simulink model "ForwardKinematic_YuMi"  (R2024a)
(part 11 of 23)

(7514214926474921*cos(q2L)*((6384186990310915*cos(q1L))/9007199254740992 + (5557241208790345*sin(q1L))/9007199254740992))/36893488147419103232 - sin(q2L)*((5557241208790345*cos(q1L))/9007199254740992 - (6384186990310915*sin(q1L))/9007199254740992)))/9007199254740992 - (1764482024691522628700660907665*sin(q3L)*((55491554575214198102159220722265*sin(q2L))/162259276829213363391578010288128 + cos(q2L)*((5557241208790345*cos(q1L))/9007199254740992 - (6384186990310915*sin(q1L))/9007199254740992) + (7514214926474921*sin(q2L)*((6384186990310915*cos(q1L))/9007199254740992 + (5557241208790345*sin(q1L))/9007199254740992))/36893488147419103232))/42535295865117307932921825928971026432))/9007199254740992))/36893488147419103232000 - (33294932745128518861295532433359*cos(q2L))/3245185536584267267831560205762560 - (81*((9007199067919185*cos(q4L))/9007199254740992 - (234819211581865*sin(q4L))/1152921504606846976)*((499823478647255911063139966257565597426350154025*sin(q2L))/1461501637330902918203684832716283019655932542976 + (9007199067919185*cos(q2L)*((5557241208790345*cos(q1L))/9007199254740992 - (6384186990310915*sin(q1L))/9007199254740992))/9007199254740992 + (67682029681889335677290557259385*sin(q2L)*((6384186990310915*cos(q1L))/9007199254740992 + (5557241208790345*sin(q1L))/9007199254740992))/332306998946228968225951765070086144))/2000 + (81222263116692158804177042061221826384594597321566869716687*((234819211581865*cos(q4L))/1152921504606846976 + (9007199067919185*sin(q4L))/9007199254740992)*((499823478647255911063139966257565597426350154025*sin(q2L))/1461501637330902918203684832716283019655932542976 + (9007199067919185*cos(q2L)*((5557241208790345*cos(q1L))/9007199254740992 - (6384186990310915*sin(q1L))/9007199254740992))/9007199254740992 + (67682029681889335677290557259385*sin(q2L)*((6384186990310915*cos(q1L))/9007199254740992 + (5557241208790345*sin(q1L))/9007199254740992))/332306998946228968225951765070086144))/306499108173177771671669405430061836723747824436720435200000 - (324259171862923063*sin(q6L)*((9007199067919185*sin(q5L)*((783310804561232573774573497517025067305577458842146606386579375*sin(q2L))/55213970774324510299478046898216203619608871777363092441300193790394368 + (14115856197532180673579726082375*cos(q2L)*((5557241208790345*cos(q1L))/9007199254740992 - (6384186990310915*sin(q1L))/9007199254740992))/340282366920938463463374607431768211456 + (106069577339469832923929692356850887620017617375*sin(q2L)*((6384186990310915*cos(q1L))/9007199254740992 + (5557241208790345*sin(q1L))/9007199254740992))/12554203470773361527671578846415332832204710888928069025792 - (234819211581865*cos(q3L)*((55491554575214198102159220722265*cos(q2L))/162259276829213363391578010288128 + (7514214926474921*cos(q2L)*((6384186990310915*cos(q1L))/9007199254740992 + (5557241208790345*sin(q1L))/9007199254740992))/36893488147419103232 - sin(q2L)*((5557241208790345*cos(q1L))/9007199254740992 - (6384186990310915*sin(q1L))/9007199254740992)))/1152921504606846976 + (67682029681889335677290557259385*cos(q3L)*((55491554575214198102159220722265*sin(q2L))/162259276829213363391578010288128 + cos(q2L)*((5557241208790345*cos(q1L))/9007199254740992 - (6384186990310915*sin(q1L))/9007199254740992) + (7514214926474921*sin(q2L)*((6384186990310915*cos(q1L))/9007199254740992 + (5557241208790345*sin(q1L))/9007199254740992))/36893488147419103232))/332306998946228968225951765070086144 - (9007199067919185*sin(q3L)*((55491554575214198102159220722265*cos(q2L))/162259276829213363391578010288128 + (7514214926474921*cos(q2L)*((6384186990310915*cos(q1L))/9007199254740992 + (5557241208790345*sin(q1L))/9007199254740992))/36893488147419103232 - sin(q2L)*((5557241208790345*cos(q1L))/9007199254740992 - (6384186990310915*sin(q1L))/9007199254740992)))/9007199254740992 - (1764482024691522628700660907665*sin(q3L)*((55491554575214198102159220722265*sin(q2L))/162259276829213363391578010288128 + cos(q2L)*((5557241208790345*cos(q1L))/9007199254740992 - (6384186990310915*sin(q1L))/9007199254740992) + (7514214926474921*sin(q2L)*((6384186990310915*cos(q1L))/9007199254740992 + (5557241208790345*sin(q1L))/9007199254740992))/36893488147419103232))/42535295865117307932921825928971026432))/9007199254740992 - cos(q5L)*(((9007199067919185*cos(q4L))/9007199254740992 - (234819211581865*sin(q4L))/1152921504606846976)*((499823478647255911063139966257565597426350154025*sin(q2L))/1461501637330902918203684832716283019655932542976 + (9007199067919185*cos(q2L)*((5557241208790345*cos(q1L))/9007199254740992 - (6384186990310915*sin(q1L))/9007199254740992))/9007199254740992 + (67682029681889335677290557259385*sin(q2L)*((6384186990310915*cos(q1L))/9007199254740992 + (5557241208790345*sin(q1L))/9007199254740992))/332306998946228968225951765070086144) + (7514214926474921*sin(q4L)*((7514214926474921*cos(q3L)*((55491554575214198102159220722265*sin(q2L))/162259276829213363391578010288128 + cos(q2L)*((5557241208790345*cos(q1L))/9007199254740992 - (6384186990310915*sin(q1L))/9007199254740992) + (7514214926474921*sin(q2L)*((6384186990310915*cos(q1L))/9007199254740992 + (5557241208790345*sin(q1L))/9007199254740992))/36893488147419103232))/36893488147419103232 - sin(q3L)*((55491554575214198102159220722265*cos(q2L))/162259276829213363391578010288128 + (7514214926474921*cos(q2L)*((6384186990310915*cos(q1L))/9007199254740992 + (5557241208790345*sin(q1L))/9007199254740992))/36893488147419103232 - sin(q2L)*((5557241208790345*cos(q1L))/9007199254740992 - (6384186990310915*sin(q1L))/9007199254740992))))/36893488147419103232 + (cos(q3L)*((55491554575214198102159220722265*cos(q2L))/162259276829213363391578010288128 + (7514214926474921*cos(q2L)*((6384186990310915*cos(q1L))/9007199254740992 + (5557241208790345*sin(q1L))/9007199254740992))/36893488147419103232 - sin(q2L)*((5557241208790345*cos(q1L))/9007199254740992 - (6384186990310915*sin(q1L))/9007199254740992)) + (7514214926474921*sin(q3L)*((55491554575214198102159220722265*sin(q2L))/162259276829213363391578010288128 + cos(q2L)*((5557241208790345*cos(q1L))/9007199254740992 - (6384186990310915*sin(q1L))/9007199254740992) + (7514214926474921*sin(q2L)*((6384186990310915*cos(q1L))/9007199254740992 + (5557241208790345*sin(q1L))/9007199254740992))/36893488147419103232))/36893488147419103232)*((7514214926474921*cos(q4L))/36893488147419103232 + (4503599440548691*sin(q4L))/4503599627370496)) + (7514214926474921*sin(q5L)*((7514214926474921*cos(q4L)*((7514214926474921*cos(q3L)*((55491554575214198102159220722265*sin(q2L))/162259276829213363391578010288128 + cos(q2L)*((5557241208790345*cos(q1L))/9007199254740992 - (6384186990310915*sin(q1L))/9007199254740992) + (7514214926474921*sin(q2L)*((6384186990310915*cos(q1L))/9007199254740992 + (5557241208790345*sin(q1L))/9007199254740992))/36893488147419103232))/36893488147419103232 - sin(q3L)*((55491554575214198102159220722265*cos(q2L))/162259276829213363391578010288128 + (7514214926474921*cos(q2L)*((6384186990310915*cos(q1L))/9007199254740992 + (5557241208790345*sin(q1L))/9007199254740992))/36893488147419103232 - sin(q2L)*((5557241208790345*cos(q1L))/9007199254740992 - (6384186990310915*sin(q1L))/9007199254740992))))/36893488147419103232 - ((234819211581865*cos(q4L))/1152921504606846976 + (9007199067919185*sin(q4L))/9007199254740992)*((499823478647255911063139966257565597426350154025*sin(q2L))/1461501637330902918203684832716283019655932542976 + (9007199067919185*cos(q2L)*((5557241208790345*cos(q1L))/9007199254740992 - (6384186990310915*sin(q1L))/9007199254740992))/9007199254740992 + (67682029681889335677290557259385*sin(q2L)*((6384186990310915*cos(q1L))/9007199254740992 + (5557241208790345*sin(q1L))/9007199254740992))/332306998946228968225951765070086144) + (cos(q3L)*((55491554575214198102159220722265*cos(q2L))/162259276829213363391578010288128 + (7514214926474921*cos(q2L)*((6384186990310915*cos(q1L))/9007199254740992 + (5557241208790345*sin(q1L))/9007199254740992))/36893488147419103232 - sin(q2L)*((5557241208790345*cos(q1L))/9007199254740992 - (6384186990310915*sin(q1L))/9007199254740992)) + (7514214926474921*sin(q3L)*((55491554575214198102159220722265*sin(q2L))/162259276829213363391578010288128 + cos(q2L)*((5557241208790345*cos(q1L))/9007199254740992 - (6384186990310915*sin(q1L))/9007199254740992) + (7514214926474921*sin(q2L)*((6384186990310915*cos(q1L))/9007199254740992 + (5557241208790345*sin(q1L))/9007199254740992))/36893488147419103232))/36893488147419103232)*((4503599440548691*cos(q4L))/4503599627370496 - (7514214926474921*sin(q4L))/36893488147419103232)))/36893488147419103232))/9007199254740992000 - (610321541873521657855151997354401418608858870661075444886782706002880706727*cos(q4L)*((7514214926474921*cos(q3L)*((55491554575214198102159220722265*sin(q2L))/162259276829213363391578010288128 + cos(q2L)*((5557241208790345*cos(q1L))/9007199254740992 - (6384186990310915*sin(q1L))/9007199254740992) + (7514214926474921*sin(q2L)*((6384186990310915*cos(q1L))/9007199254740992 + (5557241208790345*sin(q1L))/9007199254740992))/36893488147419103232))/36893488147419103232 - sin(q3L)*((55491554575214198102159220722265*cos(q2L))/162259276829213363391578010288128 + (7514214926474921*cos(q2L)*((6384186990310915*cos(q1L))/9007199254740992 + (5557241208790345*sin(q1L))/9007199254740992))/36893488147419103232 - sin(q2L)*((5557241208790345*cos(q1L))/9007199254740992 - (6384186990310915*sin(q1L))/9007199254740992))))/11307821214581659709333104004754678501295896940003961331978279688272766566400000 - (608651409044468601*sin(q4L)*((7514214926474921*cos(q3L)*((55491554575214198102159220722265*sin(q2L))/162259276829213363391578010288128 + cos(q2L)*((5557241208790345*cos(q1L))/9007199254740992 - (6384186990310915*sin(q1L))/9007199254740992) + (7514214926474921*sin(q2L)*((6384186990310915*cos(q1L))/9007199254740992 + (5557241208790345*sin(q1L))/9007199254740992))/36893488147419103232))/36893488147419103232 - sin(q3L)*((55491554575214198102159220722265*cos(q2L))/162259276829213363391578010288128 + (7514214926474921*cos(q2L)*((6384186990310915*cos(q1L))/9007199254740992 + (5557241208790345*sin(q1L))/9007199254740992))/36893488147419103232 - sin(q2L)*((5557241208790345*cos(q1L))/9007199254740992 - (6384186990310915*sin(q1L))/9007199254740992))))/73786976294838206464000 - (107465779053290185796889472867275736954369330186921663479979246519176992895505610212310958309481948671*cos(q2L)*((5557241208790345*cos(q1L))/9007199254740992 - (6384186990310915*sin(q1L))/9007199254740992))/427197407184182016479004341233910422920540904471330553989408321564443945156128110004592417387315200000 - (22542644779424763*cos(q2L)*((6384186990310915*cos(q1L))/9007199254740992 + (5557241208790345*sin(q1L))/9007199254740992))/3689348814741910323200 + (712008244765680093343103025701132101054572137019*cos(q5L)*((7514214926474921*cos(q4L)*((7514214926474921*cos(q3L)*((55491554575214198102159220722265*sin(q2L))/162259276829213363391578010288128 + cos(q2L)*((5557241208790345*cos(q1L))/9007199254740992 - (6384186990310915*sin(q1L))/9007199254740992) + (7514214926474921*sin(q2L)*((6384186990310915*cos(q1L))/9007199254740992 + (5557241208790345*sin(q1L))/9007199254740992))/36893488147419103232))/36893488147419103232 - sin(q3L)*((55491554575214198102159220722265*cos(q2L))/162259276829213363391578010288128 + (7514214926474921*cos(q2L)*((6384186990310915*cos(q1L))/9007199254740992 + (5557241208790345*sin(q1L))/9007199254740992))/36893488147419103232 - sin(q2L)*((5557241208790345*cos(q1L))/9007199254740992 - (6384186990310915*sin(q1L))/9007199254740992))))/36893488147419103232 - ((234819211581865*cos(q4L))/1152921504606846976 + (9007199067919185*sin(q4L))/9007199254740992)*((499823478647255911063139966257565597426350154025*sin(q2L))/1461501637330902918203684832716283019655932542976 + (9007199067919185*cos(q2L)*((5557241208790345*cos(q1L))/9007199254740992 - (6384186990310915*sin(q1L))/9007199254740992))/9007199254740992 + (67682029681889335677290557259385*sin(q2L)*((6384186990310915*cos(q1L))/9007199254740992 + (5557241208790345*sin(q1L))/9007199254740992))/332306998946228968225951765070086144) + (cos(q3L)*((55491554575214198102159220722265*cos(q2L))/162259276829213363391578010288128 + (7514214926474921*cos(q2L)*((6384186990310915*cos(q1L))/9007199254740992 + (5557241208790345*sin(q1L))/9007199254740992))/36893488147419103232 - sin(q2L)*((5557241208790345*cos(q1L))/9007199254740992 - (6384186990310915*sin(q1L))/9007199254740992)) + (7514214926474921*sin(q3L)*((55491554575214198102159220722265*sin(q2L))/162259276829213363391578010288128 + cos(q2L)*((5557241208790345*cos(q1L))/9007199254740992 - (6384186990310915*sin(q1L))/9007199254740992) + (7514214926474921*sin(q2L)*((6384186990310915*cos(q1L))/9007199254740992 + (5557241208790345*sin(q1L))/9007199254740992))/36893488147419103232))/36893488147419103232)*((4503599440548691*cos(q4L))/4503599627370496 - (7514214926474921*sin(q4L))/36893488147419103232)))/2451992865385422173373355243440494693789982595493763481600 + (3*sin(q2L)*((5557241208790345*cos(q1L))/9007199254740992 - (6384186990310915*sin(q1L))/9007199254740992))/100 - (807520961047489018778067709720399904923771262077295170375712179706208528987338271217011451790113918662491539890779991*sin(q2L)*((6384186990310915*cos(q1L))/9007199254740992 + (5557241208790345*sin(q1L))/9007199254740992))/15760802478557791684911616040057445522031895708186178667179317361698288708598884244565706501953966256322651196122726400000 + (27*cos(q5L)*(((9007199067919185*cos(q4L))/9007199254740992 - (234819211581865*sin(q4L))/1152921504606846976)*((499823478647255911063139966257565597426350154025*sin(q2L))/1461501637330902918203684832716283019655932542976 + (9007199067919185*cos(q2L)*((5557241208790345*cos(q1L))/9007199254740992 - (6384186990310915*sin(q1L))/9007199254740992))/9007199254740992 + (67682029681889335677290557259385*sin(q2L)*((6384186990310915*cos(q1L))/9007199254740992 + (5557241208790345*sin(q1L))/9007199254740992))/332306998946228968225951765070086144) + (7514214926474921*sin(q4L)*((7514214926474921*cos(q3L)*((55491554575214198102159220722265*sin(q2L))/162259276829213363391578010288128 + cos(q2L)*((5557241208790345*cos(q1L))/9007199254740992 - (6384186990310915*sin(q1L))/9007199254740992) + (7514214926474921*sin(q2L)*((6384186990310915*cos(q1L))/9007199254740992 + (5557241208790345*sin(q1L))/9007199254740992))/36893488147419103232))/36893488147419103232 - sin(q3L)*((55491554575214198102159220722265*cos(q2L))/162259276829213363391578010288128 + (7514214926474921*cos(q2L)*((6384186990310915*cos(q1L))/9007199254740992 + (5557241208790345*sin(q1L))/9007199254740992))/36893488147419103232 - sin(q2L)*((5557241208790345*cos(q1L))/9007199254740992 - (6384186990310915*sin(q1L))/9007199254740992))))/36893488147419103232 + (cos(q3L)*((55491554575214198102159220722265*cos(q2L))/162259276829213363391578010288128 + (7514214926474921*cos(q2L)*((6384186990310915*cos(q1L))/9007199254740992 + (5557241208790345*sin(q1L))/9007199254740992))/36893488147419103232 - sin(q2L)*((5557241208790345*cos(q1L))/9007199254740992 - (6384186990310915*sin(q1L))/9007199254740992)) + (7514214926474921*sin(q3L)*((55491554575214198102159220722265*sin(q2L))/162259276829213363391578010288128 + cos(q2L)*((5557241208790345*cos(q1L))/9007199254740992 - (6384186990310915*sin(q1L))/9007199254740992) + (7514214926474921*sin(q2L)*((6384186990310915*cos(q1L))/9007199254740992 + (5557241208790345*sin(q1L))/9007199254740992))/36893488147419103232))/36893488147419103232)*((7514214926474921*cos(q4L))/36893488147419103232 + (4503599440548691*sin(q4L))/4503599627370496)))/1000 - (202883803014822867*sin(q5L)*((7514214926474921*cos(q4L)*((7514214926474921*cos(q3L)*((55491554575214198102159220722265*sin(q2L))/162259276829213363391578010288128 + cos(q2L)*((5557241208790345*cos(q1L))/9007199254740992 - (6384186990310915*sin(q1L))/9007199254740992) + (7514214926474921*sin(q2L)*((6384186990310915*cos(q1L))/9007199254740992 + (5557241208790345*sin(q1L))/9007199254740992))/36893488147419103232))/36893488147419103232 - sin(q3L)*((55491554575214198102159220722265*cos(q2L))/162259276829213363391578010288128 + (7514214926474921*cos(q2L)*((6384186990310915*cos(q1L))/9007199254740992 + (5557241208790345*sin(q1L))/9007199254740992))/36893488147419103232 - sin(q2L)*((5557241208790345*cos(q1L))/9007199254740992 - (6384186990310915*sin(q1L))/9007199254740992))))/36893488147419103232 - ((234819211581865*cos(q4L))/1152921504606846976 + (9007199067919185*sin(q4L))/9007199254740992)*((499823478647255911063139966257565597426350154025*sin(q2L))/1461501637330902918203684832716283019655932542976 + (9007199067919185*cos(q2L)*((5557241208790345*cos(q1L))/9007199254740992 - (6384186990310915*sin(q1L))/9007199254740992))/9007199254740992 + (67682029681889335677290557259385*sin(q2L)*((6384186990310915*cos(q1L))/9007199254740992 + (5557241208790345*sin(q1L))/9007199254740992))/332306998946228968225951765070086144) + (cos(q3L)*((55491554575214198102159220722265*cos(q2L))/162259276829213363391578010288128 + (7514214926474921*cos(q2L)*((6384186990310915*cos(q1L))/9007199254740992 + (5557241208790345*sin(q1L))/9007199254740992))/36893488147419103232 - sin(q2L)*((5557241208790345*cos(q1L))/9007199254740992 - (6384186990310915*sin(q1L))/9007199254740992)) + (7514214926474921*sin(q3L)*((55491554575214198102159220722265*sin(q2L))/162259276829213363391578010288128 + cos(q2L)*((5557241208790345*cos(q1L))/9007199254740992 - (6384186990310915*sin(q1L))/9007199254740992) + (7514214926474921*sin(q2L)*((6384186990310915*cos(q1L))/9007199254740992 + (5557241208790345*sin(q1L))/9007199254740992))/36893488147419103232))/36893488147419103232)*((4503599440548691*cos(q4L))/4503599627370496 - (7514214926474921*sin(q4L))/36893488147419103232)))/36893488147419103232000 - (60617164743372705924380750591060836759586313939367162716784907429017787816377231*cos(q3L)*((55491554575214198102159220722265*cos(q2L))/162259276829213363391578010288128 + (7514214926474921*cos(q2L)*((6384186990310915*cos(q1L))/9007199254740992 + (5557241208790345*sin(q1L))/9007199254740992))/36893488147419103232 - sin(q2L)*((5557241208790345*cos(q1L))/9007199254740992 - (6384186990310915*sin(q1L))/9007199254740992)))/1447401115466452442794637312608598848165874808320507050493219800098914120499200000 + (584133382113593486367040631332731*cos(q6L)*((5885965739703093437427321469496047919878007806270640859921052774160471913354375*sin(q2L))/2037035976334486086268445688409378161051468393665936250636140449354381299763336706183397376 + (9007199067919185*((234819211581865*cos(q4L))/1152921504606846976 + (9007199067919185*sin(q4L))/9007199254740992)*((499823478647255911063139966257565597426350154025*sin(q2L))/1461501637330902918203684832716283019655932542976 + (9007199067919185*cos(q2L)*((5557241208790345*cos(q1L))/9007199254740992 - (6384186990310915*sin(q1L))/9007199254740992))/9007199254740992 + (67682029681889335677290557259385*sin(q2L)*((6384186990310915*cos(q1L))/9007199254740992 + (5557241208790345*sin(q1L))/9007199254740992))/332306998946228968225951765070086144))/9007199254740992 - (67682029681889335677290557259385*cos(q4L)*((7514214926474921*cos(q3L)*((55491554575214198102159220722265*sin(q2L))/162259276829213363391578010288128 + cos(q2L)*((5557241208790345*cos(q1L))/9007199254740992 - (6384186990310915*sin(q1L))/9007199254740992) + (7514214926474921*sin(q2L)*((6384186990310915*cos(q1L))/9007199254740992 + (5557241208790345*sin(q1L))/9007199254740992))/36893488147419103232))/36893488147419103232 - sin(q3L)*((55491554575214198102159220722265*cos(q2L))/162259276829213363391578010288128 + (7514214926474921*cos(q2L)*((6384186990310915*cos(q1L))/9007199254740992 + (5557241208790345*sin(q1L))/9007199254740992))/36893488147419103232 - sin(q2L)*((5557241208790345*cos(q1L))/9007199254740992 - (6384186990310915*sin(q1L))/9007199254740992))))/332306998946228968225951765070086144 + (106069577339469832923929692356850887620017617375*cos(q2L)*((5557241208790345*cos(q1L))/9007199254740992 - (6384186990310915*sin(q1L))/9007199254740992))/12554203470773361527671578846415332832204710888928069025792 + (797029601289130257223357069404502671534492977261568326111352375*sin(q2L)*((6384186990310915*cos(q1L))/9007199254740992 + (5557241208790345*sin(q1L))/9007199254740992))/463168356949264781694283940034751631413079938662562256157830336031652518559744 - (1764482024691522628700660907665*cos(q3L)*((55491554575214198102159220722265*cos(q2L))/162259276829213363391578010288128 + (7514214926474921*cos(q2L)*((6384186990310915*cos(q1L))/9007199254740992 + (5557241208790345*sin(q1L))/9007199254740992))/36893488147419103232 - sin(q2L)*((5557241208790345*cos(q1L))/9007199254740992 - (6384186990310915*sin(q1L))/9007199254740992)))/42535295865117307932921825928971026432 + (508577317689771495245073589786522929324694383585*cos(q3L)*((55491554575214198102159220722265*sin(q2L))/162259276829213363391578010288128 + cos(q2L)*((5557241208790345*cos(q1L))/9007199254740992 - (6384186990310915*sin(q1L))/9007199254740992) + (7514214926474921*sin(q2L)*((6384186990310915*cos(q1L))/9007199254740992 + (5557241208790345*sin(q1L))/9007199254740992))/36893488147419103232))/12259964326927110866866776217202473468949912977468817408 - (67682029681889335677290557259385*sin(q3L)*((55491554575214198102159220722265*cos(q2L))/162259276829213363391578010288128 + (7514214926474921*cos(q2L)*((6384186990310915*cos(q1L))/9007199254740992 + (5557241208790345*sin(q1L))/9007199254740992))/36893488147419103232 - sin(q2L)*((5557241208790345*cos(q1L))/9007199254740992 - (6384186990310915*sin(q1L))/9007199254740992)))/332306998946228968225951765070086144 - (13258697167433729449897784796786197386719169465*sin(q3L)*((55491554575214198102159220722265*sin(q2L))/162259276829213363391578010288128 + cos(q2L)*((5557241208790345*cos(q1L))/9007199254740992 - (6384186990310915*sin(q1L))/9007199254740992) + (7514214926474921*sin(q2L)*((6384186990310915*cos(q1L))/9007199254740992 + (5557241208790345*sin(q1L))/9007199254740992))/36893488147419103232))/1569275433846670190958947355801916604025588861116008628224 - (9007199067919185*(cos(q3L)*((55491554575214198102159220722265*cos(q2L))/162259276829213363391578010288128 + (7514214926474921*cos(q2L)*((6384186990310915*cos(q1L))/9007199254740992 + (5557241208790345*sin(q1L))/9007199254740992))/36893488147419103232 - sin(q2L)*((5557241208790345*cos(q1L))/9007199254740992 - (6384186990310915*sin(q1L))/9007199254740992)) + (7514214926474921*sin(q3L)*((55491554575214198102159220722265*sin(q2L))/162259276829213363391578010288128 + cos(q2L)*((5557241208790345*cos(q1L))/9007199254740992 - (6384186990310915*sin(q1L))/9007199254740992) + (7514214926474921*sin(q2L)*((6384186990310915*cos(q1L))/9007199254740992 + (5557241208790345*sin(q1L))/9007199254740992))/36893488147419103232))/36893488147419103232)*((4503599440548691*cos(q4L))/4503599627370496 - (7514214926474921*sin(q4L))/36893488147419103232))/9007199254740992))/16225927682921336339157801028812800 + (94754841554645069948206780163139*sin(q5L)*(((9007199067919185*cos(q4L))/9007199254740992 - (234819211581865*sin(q4L))/1152921504606846976)*((499823478647255911063139966257565597426350154025*sin(q2L))/1461501637330902918203684832716283019655932542976 + (9007199067919185*cos(q2L)*((5557241208790345*cos(q1L))/9007199254740992 - (6384186990310915*sin(q1L))/9007199254740992))/9007199254740992 + (67682029681889335677290557259385*sin(q2L)*((6384186990310915*cos(q1L))/9007199254740992 + (5557241208790345*sin(q1L))/9007199254740992))/332306998946228968225951765070086144) + (7514214926474921*sin(q4L)*((7514214926474921*cos(q3L)*((55491554575214198102159220722265*sin(q2L))/162259276829213363391578010288128 + cos(q2L)*((5557241208790345*cos(q1L))/9007199254740992 - (6384186990310915*sin(q1L))/9007199254740992) + (7514214926474921*sin(q2L)*((6384186990310915*cos(q1L))/9007199254740992 + (5557241208790345*sin(q1L))/9007199254740992))/36893488147419103232))/36893488147419103232 - sin(q3L)*((55491554575214198102159220722265*cos(q2L))/162259276829213363391578010288128 + (7514214926474921*cos(q2L)*((6384186990310915*cos(q1L))/9007199254740992 + (5557241208790345*sin(q1L))/9007199254740992))/36893488147419103232 - sin(q2L)*((5557241208790345*cos(q1L))/9007199254740992 - (6384186990310915*sin(q1L))/9007199254740992))))/36893488147419103232 + (cos(q3L)*((55491554575214198102159220722265*cos(q2L))/162259276829213363391578010288128 + (7514214926474921*cos(q2L)*((6384186990310915*cos(q1L))/9007199254740992 + (5557241208790345*sin(q1L))/9007199254740992))/36893488147419103232 - sin(q2L)*((5557241208790345*cos(q1L))/9007199254740992 - (6384186990310915*sin(q1L))/9007199254740992)) + (7514214926474921*sin(q3L)*((55491554575214198102159220722265*sin(q2L))/162259276829213363391578010288128 + cos(q2L)*((5557241208790345*cos(q1L))/9007199254740992 - (6384186990310915*sin(q1L))/9007199254740992) + (7514214926474921*sin(q2L)*((6384186990310915*cos(q1L))/9007199254740992 + (5557241208790345*sin(q1L))/9007199254740992))/36893488147419103232))/36893488147419103232)*((7514214926474921*cos(q4L))/36893488147419103232 + (4503599440548691*sin(q4L))/4503599627370496)))/66461399789245793645190353014017228800 + (347469655025336708709976918716104493695816557877713443586884917071777956519687017125887603*cos(q3L)*((55491554575214198102159220722265*sin(q2L))/162259276829213363391578010288128 + cos(q2L)*((5557241208790345*cos(q1L))/9007199254740992 - (6384186990310915*sin(q1L))/9007199254740992) + (7514214926474921*sin(q2L)*((6384186990310915*cos(q1L))/9007199254740992 + (5557241208790345*sin(q1L))/9007199254740992))/36893488147419103232))/83436993590660550093555535397248129476668145404556748826056312805555458038306271485271956520960000 - (46241644459901303158631016767207157814229090534989303509431886332469146043*sin(q3L)*((55491554575214198102159220722265*cos(q2L))/162259276829213363391578010288128 + (7514214926474921*cos(q2L)*((6384186990310915*cos(q1L))/9007199254740992 + (5557241208790345*sin(q1L))/9007199254740992))/36893488147419103232 - sin(q2L)*((5557241208790345*cos(q1L))/9007199254740992 - (6384186990310915*sin(q1L))/9007199254740992)))/2261564242916331941866620800950935700259179388000792266395655937654553313280000 + (48638874966763599*sin(q6L)*((5885965739703093437427321469496047919878007806270640859921052774160471913354375*sin(q2L))/2037035976334486086268445688409378161051468393665936250636140449354381299763336706183397376 + (9007199067919185*((234819211581865*cos(q4L))/1152921504606846976 + (9007199067919185*sin(q4L))/9007199254740992)*((499823478647255911063139966257565597426350154025*sin(q2L))/1461501637330902918203684832716283019655932542976 + (9007199067919185*cos(q2L)*((5557241208790345*cos(q1L))/9007199254740992 - (6384186990310915*sin(q1L))/9007199254740992))/9007199254740992 + (67682029681889335677290557259385*sin(q2L)*((6384186990310915*cos(q1L))/9007199254740992 + (5557241208790345*sin(q1L))/9007199254740992))/332306998946228968225951765070086144))/9007199254740992 - (67682029681889335677290557259385*cos(q4L)*((7514214926474921*cos(q3L)*((55491554575214198102159220722265*sin(q2L))/162259276829213363391578010288128 + cos(q2L)*((5557241208790345*cos(q1L))/9007199254740992 - (6384186990310915*sin(q1L))/9007199254740992) + (7514214926474921*sin(q2L)*((6384186990310915*cos(q1L))/9007199254740992 + (5557241208790345*sin(q1L))/9007199254740992))/36893488147419103232))/36893488147419103232 - sin(q3L)*((55491554575214198102159220722265*cos(q2L))/162259276829213363391578010288128 + (7514214926474921*cos(q2L)*((6384186990310915*cos(q1L))/9007199254740992 + (5557241208790345*sin(q1L))/9007199254740992))/36893488147419103232 - sin(q2L)*((5557241208790345*cos(q1L))/9007199254740992 - (6384186990310915*sin(q1L))/9007199254740992))))/332306998946228968225951765070086144 + (106069577339469832923929692356850887620017617375*cos(q2L)*((5557241208790345*cos(q1L))/9007199254740992 - (6384186990310915*sin(q1L))/9007199254740992))/12554203470773361527671578846415332832204710888928069025792 + (797029601289130257223357069404502671534492977261568326111352375*sin(q2L)*((6384186990310915*cos(q1L))/9007199254740992 + (5557241208790345*sin(q1L))/9007199254740992))/463168356949264781694283940034751631413079938662562256157830336031652518559744 - (1764482024691522628700660907665*cos(q3L)*((55491554575214198102159220722265*cos(q2L))/162259276829213363391578010288128 + (7514214926474921*cos(q2L)*((6384186990310915*cos(q1L))/9007199254740992 + (5557241208790345*sin(q1L))/9007199254740992))/36893488147419103232 - sin(q2L)*((5557241208790345*cos(q1L))/9007199254740992 - (6384186990310915*sin(q1L))/9007199254740992)))/42535295865117307932921825928971026432 + (508577317689771495245073589786522929324694383585*cos(q3L)*((55491554575214198102159220722265*sin(q2L))/162259276829213363391578010288128 + cos(q2L)*((5557241208790345*cos(q1L))/9007199254740992 - (6384186990310915*sin(q1L))/9007199254740992) + (7514214926474921*sin(q2L)*((6384186990310915*cos(q1L))/9007199254740992 + (5557241208790345*sin(q1L))/9007199254740992))/36893488147419103232))/12259964326927110866866776217202473468949912977468817408 - (67682029681889335677290557259385*sin(q3L)*((55491554575214198102159220722265*cos(q2L))/162259276829213363391578010288128 + (7514214926474921*cos(q2L)*((6384186990310915*cos(q1L))/9007199254740992 + (5557241208790345*sin(q1L))/9007199254740992))/36893488147419103232 - sin(q2L)*((5557241208790345*cos(q1L))/9007199254740992 - (6384186990310915*sin(q1L))/9007199254740992)))/332306998946228968225951765070086144 - (13258697167433729449897784796786197386719169465*sin(q3L)*((55491554575214198102159220722265*sin(q2L))/162259276829213363391578010288128 + cos(q2L)*((5557241208790345*cos(q1L))/9007199254740992 - (6384186990310915*sin(q1L))/9007199254740992) + (7514214926474921*sin(q2L)*((6384186990310915*cos(q1L))/9007199254740992 + (5557241208790345*sin(q1L))/9007199254740992))/36893488147419103232))/1569275433846670190958947355801916604025588861116008628224 - (9007199067919185*(cos(q3L)*((55491554575214198102159220722265*cos(q2L))/162259276829213363391578010288128 + (7514214926474921*cos(q2L)*((6384186990310915*cos(q1L))/9007199254740992 + (5557241208790345*sin(q1L))/9007199254740992))/36893488147419103232 - sin(q2L)*((5557241208790345*cos(q1L))/9007199254740992 - (6384186990310915*sin(q1L))/9007199254740992)) + (7514214926474921*sin(q3L)*((55491554575214198102159220722265*sin(q2L))/162259276829213363391578010288128 + cos(q2L)*((5557241208790345*cos(q1L))/9007199254740992 - (6384186990310915*sin(q1L))/9007199254740992) + (7514214926474921*sin(q2L)*((6384186990310915*cos(q1L))/9007199254740992 + (5557241208790345*sin(q1L))/9007199254740992))/36893488147419103232))/36893488147419103232)*((4503599440548691*cos(q4L))/4503599627370496 - (7514214926474921*sin(q4L))/36893488147419103232))/9007199254740992))/1801439850948198400 - (455490404115240510935077772268745492204390157443214084883134054419271951750419293234291596923751*sin(q3L)*((55491554575214198102159220722265*sin(q2L))/162259276829213363391578010288128 + cos(q2L)*((5557241208790345*cos(q1L))/9007199254740992 - (6384186990310915*sin(q1L))/9007199254740992) + (7514214926474921*sin(q2L)*((6384186990310915*cos(q1L))/9007199254740992 + (5557241208790345*sin(q1L))/9007199254740992))/36893488147419103232))/53399675898022752059875542654238802865067613058916319248676040195555493144516013750574052173414400000 - (81222263116692158804177042061221826384594597321566869716687*(cos(q3L)*((55491554575214198102159220722265*cos(q2L))/162259276829213363391578010288128 + (7514214926474921*cos(q2L)*((6384186990310915*cos(q1L))/9007199254740992 + (5557241208790345*sin(q1L))/9007199254740992))/36893488147419103232 - sin(q2L)*((5557241208790345*cos(q1L))/9007199254740992 - (6384186990310915*sin(q1L))/9007199254740992)) + (7514214926474921*sin(q3L)*((55491554575214198102159220722265*sin(q2L))/162259276829213363391578010288128 + cos(q2L)*((5557241208790345*cos(q1L))/9007199254740992 - (6384186990310915*sin(q1L))/9007199254740992) + (7514214926474921*sin(q2L)*((6384186990310915*cos(q1L))/9007199254740992 + (5557241208790345*sin(q1L))/9007199254740992))/36893488147419103232))/36893488147419103232)*((4503599440548691*cos(q4L))/4503599627370496 - (7514214926474921*sin(q4L))/36893488147419103232))/306499108173177771671669405430061836723747824436720435200000 - (81*(cos(q3L)*((55491554575214198102159220722265*cos(q2L))/162259276829213363391578010288128 + (7514214926474921*cos(q2L)*((6384186990310915*cos(q1L))/9007199254740992 + (5557241208790345*sin(q1L))/9007199254740992))/36893488147419103232 - sin(q2L)*((5557241208790345*cos(q1L))/9007199254740992 - (6384186990310915*sin(q1L))/9007199254740992)) + (7514214926474921*sin(q3L)*((55491554575214198102159220722265*sin(q2L))/162259276829213363391578010288128 + cos(q2L)*((5557241208790345*cos(q1L))/9007199254740992 - (6384186990310915*sin(q1L))/9007199254740992) + (7514214926474921*sin(q2L)*((6384186990310915*cos(q1L))/9007199254740992 + (5557241208790345*sin(q1L))/9007199254740992))/36893488147419103232))/36893488147419103232)*((7514214926474921*cos(q4L))/36893488147419103232 + (4503599440548691*sin(q4L))/4503599627370496))/2000 + (170695144106365826517608855445768431563113584343*cos(q5L)*((783310804561232573774573497517025067305577458842146606386579375*sin(q2L))/55213970774324510299478046898216203619608871777363092441300193790394368 + (14115856197532180673579726082375*cos(q2L)*((5557241208790345*cos(q1L))/9007199254740992 - (6384186990310915*sin(q1L))/9007199254740992))/340282366920938463463374607431768211456 + (106069577339469832923929692356850887620017617375*sin(q2L)*((6384186990310915*cos(q1L))/9007199254740992 + (5557241208790345*sin(q1L))/9007199254740992))/12554203470773361527671578846415332832204710888928069025792 - (234819211581865*cos(q3L)*((55491554575214198102159220722265*cos(q2L))/162259276829213363391578010288128 + (7514214926474921*cos(q2L)*((6384186990310915*cos(q1L))/9007199254740992 + (5557241208790345*sin(q1L))/9007199254740992))/36893488147419103232 - sin(q2L)*((5557241208790345*cos(q1L))/9007199254740992 - (6384186990310915*sin(q1L))/9007199254740992)))/1152921504606846976 + (67682029681889335677290557259385*cos(q3L)*((55491554575214198102159220722265*sin(q2L))/162259276829213363391578010288128 + cos(q2L)*((5557241208790345*cos(q1L))/9007199254740992 - (6384186990310915*sin(q1L))/9007199254740992) + (7514214926474921*sin(q2L)*((6384186990310915*cos(q1L))/9007199254740992 + (5557241208790345*sin(q1L))/9007199254740992))/36893488147419103232))/332306998946228968225951765070086144 - (9007199067919185*sin(q3L)*((55491554575214198102159220722265*cos(q2L))/162259276829213363391578010288128 + (7514214926474921*cos(q2L)*((6384186990310915*cos(q1L))/9007199254740992 + (5557241208790345*sin(q1L))/9007199254740992))/36893488147419103232 - sin(q2L)*((5557241208790345*cos(q1L))/9007199254740992 - (6384186990310915*sin(q1L))/9007199254740992)))/9007199254740992 - (1764482024691522628700660907665*sin(q3L)*((55491554575214198102159220722265*sin(q2L))/162259276829213363391578010288128 + cos(q2L)*((5557241208790345*cos(q1L))/9007199254740992 - (6384186990310915*sin(q1L))/9007199254740992) + (7514214926474921*sin(q2L)*((6384186990310915*cos(q1L))/9007199254740992 + (5557241208790345*sin(q1L))/9007199254740992))/36893488147419103232))/42535295865117307932921825928971026432))/119726214130147567059245861496117904970213993920593920, (48638874966763599*sin(q6L)*((9007199067919185*((4503599440548691*cos(q4L))/4503599627370496 - (7514214926474921*sin(q4L))/36893488147419103232)*((7514214926474921*cos(q3L)*((55491554575214198102159220722265*cos(q2L))/162259276829213363391578010288128 + (7514214926474921*cos(q2L)*((6384186990310915*cos(q1L))/9007199254740992 + (5557241208790345*sin(q1L))/9007199254740992))/36893488147419103232 - sin(q2L)*((5557241208790345*cos(q1L))/9007199254740992 - (6384186990310915*sin(q1L))/9007199254740992)))/36893488147419103232 + (9007199067919185*cos(q3L)*((57503643108550260546605243404275*cos(q1L))/81129638414606681695789005144064 + (50055177836018480443110068268825*sin(q1L))/81129638414606681695789005144064 - 46293577452674263141823442369649/664613997892457936451903530140172288))/9007199254740992 + sin(q3L)*((55491554575214198102159220722265*sin(q2L))/162259276829213363391578010288128 + cos(q2L)*((5557241208790345*cos(q1L))/9007199254740992 - (6384186990310915*sin(q1L))/9007199254740992) + (7514214926474921*sin(q2L)*((6384186990310915*cos(q1L))/9007199254740992 + (5557241208790345*sin(q1L))/9007199254740992))/36893488147419103232)))/9007199254740992 - (67682029681889335677290557259385*cos(q4L)*((7514214926474921*sin(q3L)*((55491554575214198102159220722265*cos(q2L))/162259276829213363391578010288128 + (7514214926474921*cos(q2L)*((6384186990310915*cos(q1L))/9007199254740992 + (5557241208790345*sin(q1L))/9007199254740992))/36893488147419103232 - sin(q2L)*((5557241208790345*cos(q1L))/9007199254740992 - (6384186990310915*sin(q1L))/9007199254740992)))/36893488147419103232 - cos(q3L)*((55491554575214198102159220722265*sin(q2L))/162259276829213363391578010288128 + cos(q2L)*((5557241208790345*cos(q1L))/9007199254740992 - (6384186990310915*sin(q1L))/9007199254740992) + (7514214926474921*sin(q2L)*((6384186990310915*cos(q1L))/9007199254740992 + (5557241208790345*sin(q1L))/9007199254740992))/36893488147419103232) + (9007199067919185*sin(q3L)*((57503643108550260546605243404275*cos(q1L))/81129638414606681695789005144064 + (50055177836018480443110068268825*sin(q1L))/81129638414606681695789005144064 - 46293577452674263141823442369649/664613997892457936451903530140172288))/9007199254740992))/332306998946228968225951765070086144 + (13258697167433729449897784796786197386719169465*cos(q3L)*((55491554575214198102159220722265*cos(q2L))/162259276829213363391578010288128 + (7514214926474921*cos(q2L)*((6384186990310915*cos(q1L))/9007199254740992 + (5557241208790345*sin(q1L))/9007199254740992))/36893488147419103232 - sin(q2L)*((5557241208790345*cos(q1L))/9007199254740992 - (6384186990310915*sin(q1L))/9007199254740992)))/1569275433846670190958947355801916604025588861116008628224 - (67682029681889335677290557259385*cos(q3L)*((55491554575214198102159220722265*sin(q2L))/162259276829213363391578010288128 + cos(q2L)*((5557241208790345*cos(q1L))/9007199254740992 - (6384186990310915*sin(q1L))/9007199254740992) + (7514214926474921*sin(q2L)*((6384186990310915*cos(q1L))/9007199254740992 + (5557241208790345*sin(q1L))/9007199254740992))/36893488147419103232))/332306998946228968225951765070086144 + (508577317689771495245073589786522929324694383585*sin(q3L)*((55491554575214198102159220722265*cos(q2L))/162259276829213363391578010288128 + (7514214926474921*cos(q2L)*((6384186990310915*cos(q1L))/9007199254740992 + (5557241208790345*sin(q1L))/9007199254740992))/36893488147419103232 - sin(q2L)*((5557241208790345*cos(q1L))/9007199254740992 - (6384186990310915*sin(q1L))/9007199254740992)))/12259964326927110866866776217202473468949912977468817408 + (15893040848161638993908057577265778144967053025*cos(q3L)*((57503643108550260546605243404275*cos(q1L))/81129638414606681695789005144064 + (50055177836018480443110068268825*sin(q1L))/81129638414606681695789005144064 - 46293577452674263141823442369649/664613997892457936451903530140172288))/383123885216472214589586756787577295904684780545900544 + (1764482024691522628700660907665*sin(q3L)*((55491554575214198102159220722265*sin(q2L))/162259276829213363391578010288128 + cos(q2L)*((5557241208790345*cos(q1L))/9007199254740992 - (6384186990310915*sin(q1L))/9007199254740992) + (7514214926474921*sin(q2L)*((6384186990310915*cos(q1L))/9007199254740992 + (5557241208790345*sin(q1L))/9007199254740992))/36893488147419103232))/42535295865117307932921825928971026432 + (609625514665592237562888769449172969868262801225*sin(q3L)*((57503643108550260546605243404275*cos(q1L))/81129638414606681695789005144064 + (50055177836018480443110068268825*sin(q1L))/81129638414606681695789005144064 - 46293577452674263141823442369649/664613997892457936451903530140172288))/2993155353253689176481146537402947624255349848014848))/1801439850948198400 - (610321541873521657855151997354401418608858870661075444886782706002880706727*cos(q4L)*((7514214926474921*sin(q3L)*((55491554575214198102159220722265*cos(q2L))/162259276829213363391578010288128 + (7514214926474921*cos(q2L)*((6384186990310915*cos(q1L))/9007199254740992 + (5557241208790345*sin(q1L))/9007199254740992))/36893488147419103232 - sin(q2L)*((5557241208790345*cos(q1L))/9007199254740992 - (6384186990310915*sin(q1L))/9007199254740992)))/36893488147419103232 - cos(q3L)*((55491554575214198102159220722265*sin(q2L))/162259276829213363391578010288128 + cos(q2L)*((5557241208790345*cos(q1L))/9007199254740992 - (6384186990310915*sin(q1L))/9007199254740992) + (7514214926474921*sin(q2L)*((6384186990310915*cos(q1L))/9007199254740992 + (5557241208790345*sin(q1L))/9007199254740992))/36893488147419103232) + (9007199067919185*sin(q3L)*((57503643108550260546605243404275*cos(q1L))/81129638414606681695789005144064 + (50055177836018480443110068268825*sin(q1L))/81129638414606681695789005144064 - 46293577452674263141823442369649/664613997892457936451903530140172288))/9007199254740992))/11307821214581659709333104004754678501295896940003961331978279688272766566400000 - (608651409044468601*sin(q4L)*((7514214926474921*sin(q3L)*((55491554575214198102159220722265*cos(q2L))/162259276829213363391578010288128 + (7514214926474921*cos(q2L)*((6384186990310915*cos(q1L))/9007199254740992 + (5557241208790345*sin(q1L))/9007199254740992))/36893488147419103232 - sin(q2L)*((5557241208790345*cos(q1L))/9007199254740992 - (6384186990310915*sin(q1L))/9007199254740992)))/36893488147419103232 - cos(q3L)*((55491554575214198102159220722265*sin(q2L))/162259276829213363391578010288128 + cos(q2L)*((5557241208790345*cos(q1L))/9007199254740992 - (6384186990310915*sin(q1L))/9007199254740992) + (7514214926474921*sin(q2L)*((6384186990310915*cos(q1L))/9007199254740992 + (5557241208790345*sin(q1L))/9007199254740992))/36893488147419103232) + (9007199067919185*sin(q3L)*((57503643108550260546605243404275*cos(q1L))/81129638414606681695789005144064 + (50055177836018480443110068268825*sin(q1L))/81129638414606681695789005144064 - 46293577452674263141823442369649/664613997892457936451903530140172288))/9007199254740992))/73786976294838206464000 + (170695144106365826517608855445768431563113584343*cos(q5L)*((1764482024691522628700660907665*cos(q3L)*((55491554575214198102159220722265*cos(q2L))/162259276829213363391578010288128 + (7514214926474921*cos(q2L)*((6384186990310915*cos(q1L))/9007199254740992 + (5557241208790345*sin(q1L))/9007199254740992))/36893488147419103232 - sin(q2L)*((5557241208790345*cos(q1L))/9007199254740992 - (6384186990310915*sin(q1L))/9007199254740992)))/42535295865117307932921825928971026432 - (9007199067919185*cos(q3L)*((55491554575214198102159220722265*sin(q2L))/162259276829213363391578010288128 + cos(q2L)*((5557241208790345*cos(q1L))/9007199254740992 - (6384186990310915*sin(q1L))/9007199254740992) + (7514214926474921*sin(q2L)*((6384186990310915*cos(q1L))/9007199254740992 + (5557241208790345*sin(q1L))/9007199254740992))/36893488147419103232))/9007199254740992 + (67682029681889335677290557259385*sin(q3L)*((55491554575214198102159220722265*cos(q2L))/162259276829213363391578010288128 + (7514214926474921*cos(q2L)*((6384186990310915*cos(q1L))/9007199254740992 + (5557241208790345*sin(q1L))/9007199254740992))/36893488147419103232 - sin(q2L)*((5557241208790345*cos(q1L))/9007199254740992 - (6384186990310915*sin(q1L))/9007199254740992)))/332306998946228968225951765070086144 + (2115063383689692319117831580025*cos(q3L)*((57503643108550260546605243404275*cos(q1L))/81129638414606681695789005144064 + (50055177836018480443110068268825*sin(q1L))/81129638414606681695789005144064 - 46293577452674263141823442369649/664613997892457936451903530140172288))/10384593717069655257060992658440192 + (234819211581865*sin(q3L)*((55491554575214198102159220722265*sin(q2L))/162259276829213363391578010288128 + cos(q2L)*((5557241208790345*cos(q1L))/9007199254740992 - (6384186990310915*sin(q1L))/9007199254740992) + (7514214926474921*sin(q2L)*((6384186990310915*cos(q1L))/9007199254740992 + (5557241208790345*sin(q1L))/9007199254740992))/36893488147419103232))/1152921504606846976 + (81129635049124235038645691064225*sin(q3L)*((57503643108550260546605243404275*cos(q1L))/81129638414606681695789005144064 + (50055177836018480443110068268825*sin(q1L))/81129638414606681695789005144064 - 46293577452674263141823442369649/664613997892457936451903530140172288))/81129638414606681695789005144064))/119726214130147567059245861496117904970213993920593920 - (48638874966763599*sin(q5L)*((1764482024691522628700660907665*cos(q3L)*((55491554575214198102159220722265*cos(q2L))/162259276829213363391578010288128 + (7514214926474921*cos(q2L)*((6384186990310915*cos(q1L))/9007199254740992 + (5557241208790345*sin(q1L))/9007199254740992))/36893488147419103232 - sin(q2L)*((5557241208790345*cos(q1L))/9007199254740992 - (6384186990310915*sin(q1L))/9007199254740992)))/42535295865117307932921825928971026432 - (9007199067919185*cos(q3L)*((55491554575214198102159220722265*sin(q2L))/162259276829213363391578010288128 + cos(q2L)*((5557241208790345*cos(q1L))/9007199254740992 - (6384186990310915*sin(q1L))/9007199254740992) + (7514214926474921*sin(q2L)*((6384186990310915*cos(q1L))/9007199254740992 + (5557241208790345*sin(q1L))/9007199254740992))/36893488147419103232))/9007199254740992 + (67682029681889335677290557259385*sin(q3L)*((55491554575214198102159220722265*cos(q2L))/162259276829213363391578010288128 + (7514214926474921*cos(q2L)*((6384186990310915*cos(q1L))/9007199254740992 + (5557241208790345*sin(q1L))/9007199254740992))/36893488147419103232 - sin(q2L)*((5557241208790345*cos(q1L))/9007199254740992 - (6384186990310915*sin(q1L))/9007199254740992)))/332306998946228968225951765070086144 + (2115063383689692319117831580025*cos(q3L)*((57503643108550260546605243404275*cos(q1L))/81129638414606681695789005144064 + (50055177836018480443110068268825*sin(q1L))/81129638414606681695789005144064 - 46293577452674263141823442369649/664613997892457936451903530140172288))/10384593717069655257060992658440192 + (234819211581865*sin(q3L)*((55491554575214198102159220722265*sin(q2L))/162259276829213363391578010288128 + cos(q2L)*((5557241208790345*cos(q1L))/9007199254740992 - (6384186990310915*sin(q1L))/9007199254740992) + (7514214926474921*sin(q2L)*((6384186990310915*cos(q1L))/9007199254740992 + (5557241208790345*sin(q1L))/9007199254740992))/36893488147419103232))/1152921504606846976 + (81129635049124235038645691064225*sin(q3L)*((57503643108550260546605243404275*cos(q1L))/81129638414606681695789005144064 + (50055177836018480443110068268825*sin(q1L))/81129638414606681695789005144064 - 46293577452674263141823442369649/664613997892457936451903530140172288))/81129638414606681695789005144064))/1801439850948198400 + (81222263116692158804177042061221826384594597321566869716687*((4503599440548691*cos(q4L))/4503599627370496 - (7514214926474921*sin(q4L))/36893488147419103232)*((7514214926474921*cos(q3L)*((55491554575214198102159220722265*cos(q2L))/162259276829213363391578010288128 + (7514214926474921*cos(q2L)*((6384186990310915*cos(q1L))/9007199254740992 + (5557241208790345*sin(q1L))/9007199254740992))/36893488147419103232 - sin(q2L)*((5557241208790345*cos(q1L))/9007199254740992 - (6384186990310915*sin(q1L))/9007199254740992)))/36893488147419103232 + (9007199067919185*cos(q3L)*((57503643108550260546605243404275*cos(q1L))/81129638414606681695789005144064 + (50055177836018480443110068268825*sin(q1L))/81129638414606681695789005144064 - 46293577452674263141823442369649/664613997892457936451903530140172288))/9007199254740992 + sin(q3L)*((55491554575214198102159220722265*sin(q2L))/162259276829213363391578010288128 + cos(q2L)*((5557241208790345*cos(q1L))/9007199254740992 - (6384186990310915*sin(q1L))/9007199254740992) + (7514214926474921*sin(q2L)*((6384186990310915*cos(q1L))/9007199254740992 + (5557241208790345*sin(q1L))/9007199254740992))/36893488147419103232)))/306499108173177771671669405430061836723747824436720435200000 + (81*((7514214926474921*cos(q4L))/36893488147419103232 + (4503599440548691*sin(q4L))/4503599627370496)*((7514214926474921*cos(q3L)*((55491554575214198102159220722265*cos(q2L))/162259276829213363391578010288128 + (7514214926474921*cos(q2L)*((6384186990310915*cos(q1L))/9007199254740992 + (5557241208790345*sin(q1L))/9007199254740992))/36893488147419103232 - sin(q2L)*((5557241208790345*cos(q1L))/9007199254740992 - (6384186990310915*sin(q1L))/9007199254740992)))/36893488147419103232 + (9007199067919185*cos(q3L)*((57503643108550260546605243404275*cos(q1L))/81129638414606681695789005144064 + (50055177836018480443110068268825*sin(q1L))/81129638414606681695789005144064 - 46293577452674263141823442369649/664613997892457936451903530140172288))/9007199254740992 + sin(q3L)*((55491554575214198102159220722265*sin(q2L))/162259276829213363391578010288128 + cos(q2L)*((5557241208790345*cos(q1L))/9007199254740992 - (6384186990310915*sin(q1L))/9007199254740992) + (7514214926474921*sin(q2L)*((6384186990310915*cos(q1L))/9007199254740992 + (5557241208790345*sin(q1L))/9007199254740992))/36893488147419103232)))/2000 + (455490404115240510935077772268745492204390157443214084883134054419271951750419293234291596923751*cos(q3L)*((55491554575214198102159220722265*cos(q2L))/162259276829213363391578010288128 + (7514214926474921*cos(q2L)*((6384186990310915*cos(q1L))/9007199254740992 + (5557241208790345*sin(q1L))/9007199254740992))/36893488147419103232 - sin(q2L)*((5557241208790345*cos(q1L))/9007199254740992 - (6384186990310915*sin(q1L))/9007199254740992)))/53399675898022752059875542654238802865067613058916319248676040195555493144516013750574052173414400000 - (2436553109258773196144549622003023*cos(q6L)*((9007199067919185*cos(q5L)*((1764482024691522628700660907665*cos(q3L)*((55491554575214198102159220722265*cos(q2L))/162259276829213363391578010288128 + (7514214926474921*cos(q2L)*((6384186990310915*cos(q1L))/9007199254740992 + (5557241208790345*sin(q1L))/9007199254740992))/36893488147419103232 - sin(q2L)*((5557241208790345*cos(q1L))/9007199254740992 - (6384186990310915*sin(q1L))/9007199254740992)))/42535295865117307932921825928971026432 - (9007199067919185*cos(q3L)*((55491554575214198102159220722265*sin(q2L))/162259276829213363391578010288128 + cos(q2L)*((5557241208790345*cos(q1L))/9007199254740992 - (6384186990310915*sin(q1L))/9007199254740992) + (7514214926474921*sin(q2L)*((6384186990310915*cos(q1L))/9007199254740992 + (5557241208790345*sin(q1L))/9007199254740992))/36893488147419103232))/9007199254740992 + (67682029681889335677290557259385*sin(q3L)*((55491554575214198102159220722265*cos(q2L))/162259276829213363391578010288128 + (7514214926474921*cos(q2L)*((6384186990310915*cos(q1L))/9007199254740992 + (5557241208790345*sin(q1L))/9007199254740992))/36893488147419103232 - sin(q2L)*((5557241208790345*cos(q1L))/9007199254740992 - (6384186990310915*sin(q1L))/9007199254740992)))/332306998946228968225951765070086144 + (2115063383689692319117831580025*cos(q3L)*((57503643108550260546605243404275*cos(q1L))/81129638414606681695789005144064 + (50055177836018480443110068268825*sin(q1L))/81129638414606681695789005144064 - 46293577452674263141823442369649/664613997892457936451903530140172288))/10384593717069655257060992658440192 + (234819211581865*sin(q3L)*((55491554575214198102159220722265*sin(q2L))/162259276829213363391578010288128 + cos(q2L)*((5557241208790345*cos(q1L))/9007199254740992 - (6384186990310915*sin(q1L))/9007199254740992) + (7514214926474921*sin(q2L)*((6384186990310915*cos(q1L))/9007199254740992 + (5557241208790345*sin(q1L))/9007199254740992))/36893488147419103232))/1152921504606846976 + (81129635049124235038645691064225*sin(q3L)*((57503643108550260546605243404275*cos(q1L))/81129638414606681695789005144064 + (50055177836018480443110068268825*sin(q1L))/81129638414606681695789005144064 - 46293577452674263141823442369649/664613997892457936451903530140172288))/81129638414606681695789005144064))/9007199254740992 + (7514214926474921*cos(q5L)*((7514214926474921*cos(q4L)*((7514214926474921*sin(q3L)*((55491554575214198102159220722265*cos(q2L))/162259276829213363391578010288128 + (7514214926474921*cos(q2L)*((6384186990310915*cos(q1L))/9007199254740992 + (5557241208790345*sin(q1L))/9007199254740992))/36893488147419103232 - sin(q2L)*((5557241208790345*cos(q1L))/9007199254740992 - (6384186990310915*sin(q1L))/9007199254740992)))/36893488147419103232 - cos(q3L)*((55491554575214198102159220722265*sin(q2L))/162259276829213363391578010288128 + cos(q2L)*((5557241208790345*cos(q1L))/9007199254740992 - (6384186990310915*sin(q1L))/9007199254740992) + (7514214926474921*sin(q2L)*((6384186990310915*cos(q1L))/9007199254740992 + (5557241208790345*sin(q1L))/9007199254740992))/36893488147419103232) + (9007199067919185*sin(q3L)*((57503643108550260546605243404275*cos(q1L))/81129638414606681695789005144064 + (50055177836018480443110068268825*sin(q1L))/81129638414606681695789005144064 - 46293577452674263141823442369649/664613997892457936451903530140172288))/9007199254740992))/36893488147419103232 - ((4503599440548691*cos(q4L))/4503599627370496 - (7514214926474921*sin(q4L))/36893488147419103232)*((7514214926474921*cos(q3L)*((55491554575214198102159220722265*cos(q2L))/162259276829213363391578010288128 + (7514214926474921*cos(q2L)*((6384186990310915*cos(q1L))/9007199254740992 + (5557241208790345*sin(q1L))/9007199254740992))/36893488147419103232 - sin(q2L)*((5557241208790345*cos(q1L))/9007199254740992 - (6384186990310915*sin(q1L))/9007199254740992)))/36893488147419103232 + (9007199067919185*cos(q3L)*((57503643108550260546605243404275*cos(q1L))/81129638414606681695789005144064 + (50055177836018480443110068268825*sin(q1L))/81129638414606681695789005144064 - 46293577452674263141823442369649/664613997892457936451903530140172288))/9007199254740992 + sin(q3L)*((55491554575214198102159220722265*sin(q2L))/162259276829213363391578010288128 + cos(q2L)*((5557241208790345*cos(q1L))/9007199254740992 - (6384186990310915*sin(q1L))/9007199254740992) + (7514214926474921*sin(q2L)*((6384186990310915*cos(q1L))/9007199254740992 + (5557241208790345*sin(q1L))/9007199254740992))/36893488147419103232))))/36893488147419103232 + sin(q5L)*((7514214926474921*sin(q4L)*((7514214926474921*sin(q3L)*((55491554575214198102159220722265*cos(q2L))/162259276829213363391578010288128 + (7514214926474921*cos(q2L)*((6384186990310915*cos(q1L))/9007199254740992 + (5557241208790345*sin(q1L))/9007199254740992))/36893488147419103232 - sin(q2L)*((5557241208790345*cos(q1L))/9007199254740992 - (6384186990310915*sin(q1L))/9007199254740992)))/36893488147419103232 - cos(q3L)*((55491554575214198102159220722265*sin(q2L))/162259276829213363391578010288128 + cos(q2L)*((5557241208790345*cos(q1L))/9007199254740992 - (6384186990310915*sin(q1L))/9007199254740992) + (7514214926474921*sin(q2L)*((6384186990310915*cos(q1L))/9007199254740992 + (5557241208790345*sin(q1L))/9007199254740992))/36893488147419103232) + (9007199067919185*sin(q3L)*((57503643108550260546605243404275*cos(q1L))/81129638414606681695789005144064 + (50055177836018480443110068268825*sin(q1L))/81129638414606681695789005144064 - 46293577452674263141823442369649/664613997892457936451903530140172288))/9007199254740992))/36893488147419103232 - ((7514214926474921*cos(q4L))/36893488147419103232 + (4503599440548691*sin(q4L))/4503599627370496)*((7514214926474921*cos(q3L)*((55491554575214198102159220722265*cos(q2L))/162259276829213363391578010288128 + (7514214926474921*cos(q2L)*((6384186990310915*cos(q1L))/9007199254740992 + (5557241208790345*sin(q1L))/9007199254740992))/36893488147419103232 - sin(q2L)*((5557241208790345*cos(q1L))/9007199254740992 - (6384186990310915*sin(q1L))/9007199254740992)))/36893488147419103232 + (9007199067919185*cos(q3L)*((57503643108550260546605243404275*cos(q1L))/81129638414606681695789005144064 + (50055177836018480443110068268825*sin(q1L))/81129638414606681695789005144064 - 46293577452674263141823442369649/664613997892457936451903530140172288))/9007199254740992 + sin(q3L)*((55491554575214198102159220722265*sin(q2L))/162259276829213363391578010288128 + cos(q2L)*((5557241208790345*cos(q1L))/9007199254740992 - (6384186990310915*sin(q1L))/9007199254740992) + (7514214926474921*sin(q2L)*((6384186990310915*cos(q1L))/9007199254740992 + (5557241208790345*sin(q1L))/9007199254740992))/36893488147419103232)))))/332306998946228968225951765070086144000 + (712008244765680093343103025701132101054572137019*cos(q5L)*((7514214926474921*cos(q4L)*((7514214926474921*sin(q3L)*((55491554575214198102159220722265*cos(q2L))/162259276829213363391578010288128 + (7514214926474921*cos(q2L)*((6384186990310915*cos(q1L))/9007199254740992 + (5557241208790345*sin(q1L))/9007199254740992))/36893488147419103232 - sin(q2L)*((5557241208790345*cos(q1L))/9007199254740992 - (6384186990310915*sin(q1L))/9007199254740992)))/36893488147419103232 - cos(q3L)*((55491554575214198102159220722265*sin(q2L))/162259276829213363391578010288128 + cos(q2L)*((5557241208790345*cos(q1L))/9007199254740992 - (6384186990310915*sin(q1L))/9007199254740992) + (7514214926474921*sin(q2L)*((6384186990310915*cos(q1L))/9007199254740992 + (5557241208790345*sin(q1L))/9007199254740992))/36893488147419103232) + (9007199067919185*sin(q3L)*((57503643108550260546605243404275*cos(q1L))/81129638414606681695789005144064 + (50055177836018480443110068268825*sin(q1L))/81129638414606681695789005144064 - 46293577452674263141823442369649/664613997892457936451903530140172288))/9007199254740992))/36893488147419103232 - ((4503599440548691*cos(q4L))/4503599627370496 - (7514214926474921*sin(q4L))/36893488147419103232)*((7514214926474921*cos(q3L)*((55491554575214198102159220722265*cos(q2L))/162259276829213363391578010288128 + (7514214926474921*cos(q2L)*((6384186990310915*cos(q1L))/9007199254740992 + (5557241208790345*sin(q1L))/9007199254740992))/36893488147419103232 - sin(q2L)*((5557241208790345*cos(q1L))/9007199254740992 - (6384186990310915*sin(q1L))/9007199254740992)))/36893488147419103232 + (9007199067919185*cos(q3L)*((57503643108550260546605243404275*cos(q1L))/81129638414606681695789005144064 + (50055177836018480443110068268825*sin(q1L))/81129638414606681695789005144064 - 46293577452674263141823442369649/664613997892457936451903530140172288))/9007199254740992 + sin(q3L)*((55491554575214198102159220722265*sin(q2L))/162259276829213363391578010288128 + cos(q2L)*((5557241208790345*cos(q1L))/9007199254740992 - (6384186990310915*sin(q1L))/9007199254740992) + (7514214926474921*sin(q2L)*((6384186990310915*cos(q1L))/9007199254740992 + (5557241208790345*sin(q1L))/9007199254740992))/36893488147419103232))))/2451992865385422173373355243440494693789982595493763481600 - (46241644459901303158631016767207157814229090534989303509431886332469146043*cos(q3L)*((55491554575214198102159220722265*sin(q2L))/162259276829213363391578010288128 + cos(q2L)*((5557241208790345*cos(q1L))/9007199254740992 - (6384186990310915*sin(q1L))/9007199254740992) + (7514214926474921*sin(q2L)*((6384186990310915*cos(q1L))/9007199254740992 + (5557241208790345*sin(q1L))/9007199254740992))/36893488147419103232))/2261564242916331941866620800950935700259179388000792266395655937654553313280000 + (347469655025336708709976918716104493695816557877713443586884917071777956519687017125887603*sin(q3L)*((55491554575214198102159220722265*cos(q2L))/162259276829213363391578010288128 + (7514214926474921*cos(q2L)*((6384186990310915*cos(q1L))/9007199254740992 + (5557241208790345*sin(q1L))/9007199254740992))/36893488147419103232 - sin(q2L)*((5557241208790345*cos(q1L))/9007199254740992 - (6384186990310915*sin(q1L))/9007199254740992)))/83436993590660550093555535397248129476668145404556748826056312805555458038306271485271956520960000 - (202883803014822867*sin(q6L)*((9007199067919185*cos(q5L)*((1764482024691522628700660907665*cos(q3L)*((55491554575214198102159220722265*cos(q2L))/162259276829213363391578010288128 + (7514214926474921*cos(q2L)*((6384186990310915*cos(q1L))/9007199254740992 + (5557241208790345*sin(q1L))/9007199254740992))/36893488147419103232 - sin(q2L)*((5557241208790345*cos(q1L))/9007199254740992 - (6384186990310915*sin(q1L))/9007199254740992)))/42535295865117307932921825928971026432 - (9007199067919185*cos(q3L)*((55491554575214198102159220722265*sin(q2L))/162259276829213363391578010288128 + cos(q2L)*((5557241208790345*cos(q1L))/9007199254740992 - (6384186990310915*sin(q1L))/9007199254740992) + (7514214926474921*sin(q2L)*((6384186990310915*cos(q1L))/9007199254740992 + (5557241208790345*sin(q1L))/9007199254740992))/36893488147419103232))/9007199254740992 + (67682029681889335677290557259385*sin(q3L)*((55491554575214198102159220722265*cos(q2L))/162259276829213363391578010288128 + (7514214926474921*cos(q2L)*((6384186990310915*cos(q1L))/9007199254740992 + (5557241208790345*sin(q1L))/9007199254740992))/36893488147419103232 - sin(q2L)*((5557241208790345*cos(q1L))/9007199254740992 - (6384186990310915*sin(q1L))/9007199254740992)))/332306998946228968225951765070086144 + (2115063383689692319117831580025*cos(q3L)*((57503643108550260546605243404275*cos(q1L))/81129638414606681695789005144064 + (50055177836018480443110068268825*sin(q1L))/81129638414606681695789005144064 - 46293577452674263141823442369649/664613997892457936451903530140172288))/10384593717069655257060992658440192 + (234819211581865*sin(q3L)*((55491554575214198102159220722265*sin(q2L))/162259276829213363391578010288128 + cos(q2L)*((5557241208790345*cos(q1L))/9007199254740992 - (6384186990310915*sin(q1L))/9007199254740992) + (7514214926474921*sin(q2L)*((6384186990310915*cos(q1L))/9007199254740992 + (5557241208790345*sin(q1L))/9007199254740992))/36893488147419103232))/1152921504606846976 + (81129635049124235038645691064225*sin(q3L)*((57503643108550260546605243404275*cos(q1L))/81129638414606681695789005144064 + (50055177836018480443110068268825*sin(q1L))/81129638414606681695789005144064 - 46293577452674263141823442369649/664613997892457936451903530140172288))/81129638414606681695789005144064))/9007199254740992 + (7514214926474921*cos(q5L)*((7514214926474921*cos(q4L)*((7514214926474921*sin(q3L)*((55491554575214198102159220722265*cos(q2L))/162259276829213363391578010288128 + (7514214926474921*cos(q2L)*((6384186990310915*cos(q1L))/9007199254740992 + (5557241208790345*sin(q1L))/9007199254740992))/36893488147419103232 - sin(q2L)*((5557241208790345*cos(q1L))/9007199254740992 - (6384186990310915*sin(q1L))/9007199254740992)))/36893488147419103232 - cos(q3L)*((55491554575214198102159220722265*sin(q2L))/162259276829213363391578010288128 + cos(q2L)*((5557241208790345*cos(q1L))/9007199254740992 - (6384186990310915*sin(q1L))/9007199254740992) + (7514214926474921*sin(q2L)*((6384186990310915*cos(q1L))/9007199254740992 + (5557241208790345*sin(q1L))/9007199254740992))/36893488147419103232) + (9007199067919185*sin(q3L)*((57503643108550260546605243404275*cos(q1L))/81129638414606681695789005144064 + (50055177836018480443110068268825*sin(q1L))/81129638414606681695789005144064 - 46293577452674263141823442369649/664613997892457936451903530140172288))/9007199254740992))/36893488147419103232 - ((4503599440548691*cos(q4L))/4503599627370496 - (7514214926474921*sin(q4L))/36893488147419103232)*((7514214926474921*cos(q3L)*((55491554575214198102159220722265*cos(q2L))/162259276829213363391578010288128 + (7514214926474921*cos(q2L)*((6384186990310915*cos(q1L))/9007199254740992 + (5557241208790345*sin(q1L))/9007199254740992))/36893488147419103232 - sin(q2L)*((5557241208790345*cos(q1L))/9007199254740992 - (6384186990310915*sin(q1L))/9007199254740992)))/36893488147419103232 + (9007199067919185*cos(q3L)*((57503643108550260546605243404275*cos(q1L))/81129638414606681695789005144064 + (50055177836018480443110068268825*sin(q1L))/81129638414606681695789005144064 - 46293577452674263141823442369649/664613997892457936451903530140172288))/9007199254740992 + sin(q3L)*((55491554575214198102159220722265*sin(q2L))/162259276829213363391578010288128 + cos(q2L)*((5557241208790345*cos(q1L))/9007199254740992 - (6384186990310915*sin(q1L))/9007199254740992) + (7514214926474921*sin(q2L)*((6384186990310915*cos(q1L))/9007199254740992 + (5557241208790345*sin(q1L))/9007199254740992))/36893488147419103232))))/36893488147419103232 + sin(q5L)*((7514214926474921*sin(q4L)*((7514214926474921*sin(q3L)*((55491554575214198102159220722265*cos(q2L))/162259276829213363391578010288128 + (7514214926474921*cos(q2L)*((6384186990310915*cos(q1L))/9007199254740992 + (5557241208790345*sin(q1L))/9007199254740992))/36893488147419103232 - sin(q2L)*((5557241208790345*cos(q1L))/9007199254740992 - (6384186990310915*sin(q1L))/9007199254740992)))/36893488147419103232 - cos(q3L)*((55491554575214198102159220722265*sin(q2L))/162259276829213363391578010288128 + cos(q2L)*((5557241208790345*cos(q1L))/9007199254740992 - (6384186990310915*sin(q1L))/9007199254740992) + (7514214926474921*sin(q2L)*((6384186990310915*cos(q1L))/9007199254740992 + (5557241208790345*sin(q1L))/9007199254740992))/36893488147419103232) + (9007199067919185*sin(q3L)*((57503643108550260546605243404275*cos(q1L))/81129638414606681695789005144064 + (50055177836018480443110068268825*sin(q1L))/81129638414606681695789005144064 - 46293577452674263141823442369649/664613997892457936451903530140172288))/9007199254740992))/36893488147419103232 - ((7514214926474921*cos(q4L))/36893488147419103232 + (4503599440548691*sin(q4L))/4503599627370496)*((7514214926474921*cos(q3L)*((55491554575214198102159220722265*cos(q2L))/162259276829213363391578010288128 + (7514214926474921*cos(q2L)*((6384186990310915*cos(q1L))/9007199254740992 + (5557241208790345*sin(q1L))/9007199254740992))/36893488147419103232 - sin(q2L)*((5557241208790345*cos(q1L))/9007199254740992 - (6384186990310915*sin(q1L))/9007199254740992)))/36893488147419103232 + (9007199067919185*cos(q3L)*((57503643108550260546605243404275*cos(q1L))/81129638414606681695789005144064 + (50055177836018480443110068268825*sin(q1L))/81129638414606681695789005144064 - 46293577452674263141823442369649/664613997892457936451903530140172288))/9007199254740992 + sin(q3L)*((55491554575214198102159220722265*sin(q2L))/162259276829213363391578010288128 + cos(q2L)*((5557241208790345*cos(q1L))/9007199254740992 - (6384186990310915*sin(q1L))/9007199254740992) + (7514214926474921*sin(q2L)*((6384186990310915*cos(q1L))/9007199254740992 + (5557241208790345*sin(q1L))/9007199254740992))/36893488147419103232)))))/36893488147419103232000 + (27*cos(q6L)*((9007199067919185*sin(q5L)*((1764482024691522628700660907665*cos(q3L)*((55491554575214198102159220722265*cos(q2L))/162259276829213363391578010288128 + (7514214926474921*cos(q2L)*((6384186990310915*cos(q1L))/9007199254740992 + (5557241208790345*sin(q1L))/9007199254740992))/36893488147419103232 - sin(q2L)*((5557241208790345*cos(q1L))/9007199254740992 - (6384186990310915*sin(q1L))/9007199254740992)))/42535295865117307932921825928971026432 - (9007199067919185*cos(q3L)*((55491554575214198102159220722265*sin(q2L))/162259276829213363391578010288128 + cos(q2L)*((5557241208790345*cos(q1L))/9007199254740992 - (6384186990310915*sin(q1L))/9007199254740992) + (7514214926474921*sin(q2L)*((6384186990310915*cos(q1L))/9007199254740992 + (5557241208790345*sin(q1L))/9007199254740992))/36893488147419103232))/9007199254740992 + (67682029681889335677290557259385*sin(q3L)*((55491554575214198102159220722265*cos(q2L))/162259276829213363391578010288128 + (7514214926474921*cos(q2L)*((6384186990310915*cos(q1L))/9007199254740992 + (5557241208790345*sin(q1L))/9007199254740992))/36893488147419103232 - sin(q2L)*((5557241208790345*cos(q1L))/9007199254740992 - (6384186990310915*sin(q1L))/9007199254740992)))/332306998946228968225951765070086144 + (2115063383689692319117831580025*cos(q3L)*((57503643108550260546605243404275*cos(q1L))/81129638414606681695789005144064 + (50055177836018480443110068268825*sin(q1L))/81129638414606681695789005144064 - 46293577452674263141823442369649/664613997892457936451903530140172288))/10384593717069655257060992658440192 + (234819211581865*sin(q3L)*((55491554575214198102159220722265*sin(q2L))/162259276829213363391578010288128 + cos(q2L)*((5557241208790345*cos(q1L))/9007199254740992 - (6384186990310915*sin(q1L))/9007199254740992) + (7514214926474921*sin(q2L)*((6384186990310915*cos(q1L))/9007199254740992 + (5557241208790345*sin(q1L))/9007199254740992))/36893488147419103232))/1152921504606846976 + (81129635049124235038645691064225*sin(q3L)*((57503643108550260546605243404275*cos(q1L))/81129638414606681695789005144064 + (50055177836018480443110068268825*sin(q1L))/81129638414606681695789005144064 - 46293577452674263141823442369649/664613997892457936451903530140172288))/81129638414606681695789005144064))/9007199254740992 - cos(q5L)*((7514214926474921*sin(q4L)*((7514214926474921*sin(q3L)*((55491554575214198102159220722265*cos(q2L))/162259276829213363391578010288128 + (7514214926474921*cos(q2L)*((6384186990310915*cos(q1L))/9007199254740992 + (5557241208790345*sin(q1L))/9007199254740992))/36893488147419103232 - sin(q2L)*((5557241208790345*cos(q1L))/9007199254740992 - (6384186990310915*sin(q1L))/9007199254740992)))/36893488147419103232 - cos(q3L)*((55491554575214198102159220722265*sin(q2L))/162259276829213363391578010288128 + cos(q2L)*((5557241208790345*cos(q1L))/9007199254740992 - (6384186990310915*sin(q1L))/9007199254740992) + (7514214926474921*sin(q2L)*((6384186990310915*cos(q1L))/9007199254740992 + (5557241208790345*sin(q1L))/9007199254740992))/36893488147419103232) + (9007199067919185*sin(q3L)*((57503643108550260546605243404275*cos(q1L))/81129638414606681695789005144064 + (50055177836018480443110068268825*sin(q1L))/81129638414606681695789005144064 - 46293577452674263141823442369649/664613997892457936451903530140172288))/9007199254740992))/36893488147419103232 - ((7514214926474921*cos(q4L))/36893488147419103232 + (4503599440548691*sin(q4L))/4503599627370496)*((7514214926474921*cos(q3L)*((55491554575214198102159220722265*cos(q2L))/162259276829213363391578010288128 + (7514214926474921*cos(q2L)*((6384186990310915*cos(q1L))/9007199254740992 + (5557241208790345*sin(q1L))/9007199254740992))/36893488147419103232 - sin(q2L)*((5557241208790345*cos(q1L))/9007199254740992 - (6384186990310915*sin(q1L))/9007199254740992)))/36893488147419103232 + (9007199067919185*cos(q3L)*((57503643108550260546605243404275*cos(q1L))/81129638414606681695789005144064 + (50055177836018480443110068268825*sin(q1L))/81129638414606681695789005144064 - 46293577452674263141823442369649/664613997892457936451903530140172288))/9007199254740992 + sin(q3L)*((55491554575214198102159220722265*sin(q2L))/162259276829213363391578010288128 + cos(q2L)*((5557241208790345*cos(q1L))/9007199254740992 - (6384186990310915*sin(q1L))/9007199254740992) + (7514214926474921*sin(q2L)*((6384186990310915*cos(q1L))/9007199254740992 + (5557241208790345*sin(q1L))/9007199254740992))/36893488147419103232))) + (7514214926474921*sin(q5L)*((7514214926474921*cos(q4L)*((7514214926474921*sin(q3L)*((55491554575214198102159220722265*cos(q2L))/162259276829213363391578010288128 + (7514214926474921*cos(q2L)*((6384186990310915*cos(q1L))/9007199254740992 + (5557241208790345*sin(q1L))/9007199254740992))/36893488147419103232 - sin(q2L)*((5557241208790345*cos(q1L))/9007199254740992 - (6384186990310915*sin(q1L))/9007199254740992)))/36893488147419103232 - cos(q3L)*((55491554575214198102159220722265*sin(q2L))/162259276829213363391578010288128 + cos(q2L)*((5557241208790345*cos(q1L))/9007199254740992 - (6384186990310915*sin(q1L))/9007199254740992) + (7514214926474921*sin(q2L)*((6384186990310915*cos(q1L))/9007199254740992 + (5557241208790345*sin(q1L))/9007199254740992))/36893488147419103232) + (9007199067919185*sin(q3L)*((57503643108550260546605243404275*cos(q1L))/81129638414606681695789005144064 + (50055177836018480443110068268825*sin(q1L))/81129638414606681695789005144064 - 46293577452674263141823442369649/664613997892457936451903530140172288))/9007199254740992))/36893488147419103232 - ((4503599440548691*cos(q4L))/4503599627370496 - (7514214926474921*sin(q4L))/36893488147419103232)*((7514214926474921*cos(q3L)*((55491554575214198102159220722265*cos(q2L))/162259276829213363391578010288128 + (7514214926474921*cos(q2L)*((6384186990310915*cos(q1L))/9007199254740992 + (5557241208790345*sin(q1L))/9007199254740992))/36893488147419103232 - sin(q2L)*((5557241208790345*cos(q1L))/9007199254740992 - (6384186990310915*sin(q1L))/9007199254740992)))/36893488147419103232 + (9007199067919185*cos(q3L)*((57503643108550260546605243404275*cos(q1L))/81129638414606681695789005144064 + (50055177836018480443110068268825*sin(q1L))/81129638414606681695789005144064 - 46293577452674263141823442369649/664613997892457936451903530140172288))/9007199254740992 + sin(q3L)*((55491554575214198102159220722265*sin(q2L))/162259276829213363391578010288128 + cos(q2L)*((5557241208790345*cos(q1L))/9007199254740992 - (6384186990310915*sin(q1L))/9007199254740992) + (7514214926474921*sin(q2L)*((6384186990310915*cos(q1L))/9007199254740992 + (5557241208790345*sin(q1L))/9007199254740992))/36893488147419103232))))/36893488147419103232))/1000 + (109198173955282063961996941994332957526645881091499469714283881779231664456243735535448036415347*cos(q3L)*((57503643108550260546605243404275*cos(q1L))/81129638414606681695789005144064 + (50055177836018480443110068268825*sin(q1L))/81129638414606681695789005144064 - 46293577452674263141823442369649/664613997892457936451903530140172288))/2607406049708142190423610481164004046145879543892398400814259775173608063697070983914748641280000 + (27*cos(q5L)*((7514214926474921*sin(q4L)*((7514214926474921*sin(q3L)*((55491554575214198102159220722265*cos(q2L))/162259276829213363391578010288128 + (7514214926474921*cos(q2L)*((6384186990310915*cos(q1L))/9007199254740992 + (5557241208790345*sin(q1L))/9007199254740992))/36893488147419103232 - sin(q2L)*((5557241208790345*cos(q1L))/9007199254740992 - (6384186990310915*sin(q1L))/9007199254740992)))/36893488147419103232 - cos(q3L)*((55491554575214198102159220722265*sin(q2L))/162259276829213363391578010288128 + cos(q2L)*((5557241208790345*cos(q1L))/9007199254740992 - (6384186990310915*sin(q1L))/9007199254740992) + (7514214926474921*sin(q2L)*((6384186990310915*cos(q1L))/9007199254740992 + (5557241208790345*sin(q1L))/9007199254740992))/36893488147419103232) + (9007199067919185*sin(q3L)*((57503643108550260546605243404275*cos(q1L))/81129638414606681695789005144064 + (50055177836018480443110068268825*sin(q1L))/81129638414606681695789005144064 - 46293577452674263141823442369649/664613997892457936451903530140172288))/9007199254740992))/36893488147419103232 - ((7514214926474921*cos(q4L))/36893488147419103232 + (4503599440548691*sin(q4L))/4503599627370496)*((7514214926474921*cos(q3L)*((55491554575214198102159220722265*cos(q2L))/162259276829213363391578010288128 + (7514214926474921*cos(q2L)*((6384186990310915*cos(q1L))/9007199254740992 + (5557241208790345*sin(q1L))/9007199254740992))/36893488147419103232 - sin(q2L)*((5557241208790345*cos(q1L))/9007199254740992 - (6384186990310915*sin(q1L))/9007199254740992)))/36893488147419103232 + (9007199067919185*cos(q3L)*((57503643108550260546605243404275*cos(q1L))/81129638414606681695789005144064 + (50055177836018480443110068268825*sin(q1L))/81129638414606681695789005144064 - 46293577452674263141823442369649/664613997892457936451903530140172288))/9007199254740992 + sin(q3L)*((55491554575214198102159220722265*sin(q2L))/162259276829213363391578010288128 + cos(q2L)*((5557241208790345*cos(q1L))/9007199254740992 - (6384186990310915*sin(q1L))/9007199254740992) + (7514214926474921*sin(q2L)*((6384186990310915*cos(q1L))/9007199254740992 + (5557241208790345*sin(q1L))/9007199254740992))/36893488147419103232))))/1000 - (202883803014822867*sin(q5L)*((7514214926474921*cos(q4L)*((7514214926474921*sin(q3L)*((55491554575214198102159220722265*cos(q2L))/162259276829213363391578010288128 + (7514214926474921*cos(q2L)*((6384186990310915*cos(q1L))/9007199254740992 + (5557241208790345*sin(q1L))/9007199254740992))/36893488147419103232 - sin(q2L)*((5557241208790345*cos(q1L))/9007199254740992 - (6384186990310915*sin(q1L))/9007199254740992)))/36893488147419103232 - cos(q3L)*((55491554575214198102159220722265*sin(q2L))/162259276829213363391578010288128 + cos(q2L)*((5557241208790345*cos(q1L))/9007199254740992 - (6384186990310915*sin(q1L))/9007199254740992) + (7514214926474921*sin(q2L)*((6384186990310915*cos(q1L))/9007199254740992 + (5557241208790345*sin(q1L))/9007199254740992))/36893488147419103232) + (9007199067919185*sin(q3L)*((57503643108550260546605243404275*cos(q1L))/81129638414606681695789005144064 + (50055177836018480443110068268825*sin(q1L))/81129638414606681695789005144064 - 46293577452674263141823442369649/664613997892457936451903530140172288))/9007199254740992))/36893488147419103232 - ((4503599440548691*cos(q4L))/4503599627370496 - (7514214926474921*sin(q4L))/36893488147419103232)*((7514214926474921*cos(q3L)*((55491554575214198102159220722265*cos(q2L))/162259276829213363391578010288128 + (7514214926474921*cos(q2L)*((6384186990310915*cos(q1L))/9007199254740992 + (5557241208790345*sin(q1L))/9007199254740992))/36893488147419103232 - sin(q2L)*((5557241208790345*cos(q1L))/9007199254740992 - (6384186990310915*sin(q1L))/9007199254740992)))/36893488147419103232 + (9007199067919185*cos(q3L)*((57503643108550260546605243404275*cos(q1L))/81129638414606681695789005144064 + (50055177836018480443110068268825*sin(q1L))/81129638414606681695789005144064 - 46293577452674263141823442369649/664613997892457936451903530140172288))/9007199254740992 + sin(q3L)*((55491554575214198102159220722265*sin(q2L))/162259276829213363391578010288128 + cos(q2L)*((5557241208790345*cos(q1L))/9007199254740992 - (6384186990310915*sin(q1L))/9007199254740992) + (7514214926474921*sin(q2L)*((6384186990310915*cos(q1L))/9007199254740992 + (5557241208790345*sin(q1L))/9007199254740992))/36893488147419103232))))/36893488147419103232000 + (60617164743372705924380750591060836759586313939367162716784907429017787816377231*sin(q3L)*((55491554575214198102159220722265*sin(q2L))/162259276829213363391578010288128 + cos(q2L)*((5557241208790345*cos(q1L))/9007199254740992 - (6384186990310915*sin(q1L))/9007199254740992) + (7514214926474921*sin(q2L)*((6384186990310915*cos(q1L))/9007199254740992 + (5557241208790345*sin(q1L))/9007199254740992))/36893488147419103232))/1447401115466452442794637312608598848165874808320507050493219800098914120499200000 - (324259171862923063*sin(q6L)*((9007199067919185*sin(q5L)*((1764482024691522628700660907665*cos(q3L)*((55491554575214198102159220722265*cos(q2L))/162259276829213363391578010288128 + (7514214926474921*cos(q2L)*((6384186990310915*cos(q1L))/9007199254740992 + (5557241208790345*sin(q1L))/9007199254740992))/36893488147419103232 - sin(q2L)*((5557241208790345*cos(q1L))/9007199254740992 - (6384186990310915*sin(q1L))/9007199254740992)))/42535295865117307932921825928971026432 - (9007199067919185*cos(q3L)*((55491554575214198102159220722265*sin(q2L))/162259276829213363391578010288128 + cos(q2L)*((5557241208790345*cos(q1L))/9007199254740992 - (6384186990310915*sin(q1L))/9007199254740992) + (7514214926474921*sin(q2L)*((6384186990310915*cos(q1L))/9007199254740992 + (5557241208790345*sin(q1L))/9007199254740992))/36893488147419103232))/9007199254740992 + (67682029681889335677290557259385*sin(q3L)*((55491554575214198102159220722265*cos(q2L))/162259276829213363391578010288128 + (7514214926474921*cos(q2L)*((6384186990310915*cos(q1L))/9007199254740992 + (5557241208790345*sin(q1L))/9007199254740992))/36893488147419103232 - sin(q2L)*((5557241208790345*cos(q1L))/9007199254740992 - (6384186990310915*sin(q1L))/9007199254740992)))/332306998946228968225951765070086144 + (2115063383689692319117831580025*cos(q3L)*((57503643108550260546605243404275*cos(q1L))/81129638414606681695789005144064 + (50055177836018480443110068268825*sin(q1L))/81129638414606681695789005144064 - 46293577452674263141823442369649/664613997892457936451903530140172288))/10384593717069655257060992658440192 + (234819211581865*sin(q3L)*((55491554575214198102159220722265*sin(q2L))/162259276829213363391578010288128 + cos(q2L)*((5557241208790345*cos(q1L))/9007199254740992 - (6384186990310915*sin(q1L))/9007199254740992) + (7514214926474921*sin(q2L)*((6384186990310915*cos(q1L))/9007199254740992 + (5557241208790345*sin(q1L))/9007199254740992))/36893488147419103232))/1152921504606846976 + (81129635049124235038645691064225*sin(q3L)*((57503643108550260546605243404275*cos(q1L))/81129638414606681695789005144064 + (50055177836018480443110068268825*sin(q1L))/81129638414606681695789005144064 - 46293577452674263141823442369649/664613997892457936451903530140172288))/81129638414606681695789005144064))/9007199254740992 - cos(q5L)*((7514214926474921*sin(q4L)*((7514214926474921*sin(q3L)*((55491554575214198102159220722265*cos(q2L))/162259276829213363391578010288128 + (7514214926474921*cos(q2L)*((6384186990310915*cos(q1L))/9007199254740992 + (5557241208790345*sin(q1L))/9007199254740992))/36893488147419103232 - sin(q2L)*((5557241208790345*cos(q1L))/9007199254740992 - (6384186990310915*sin(q1L))/9007199254740992)))/36893488147419103232 - cos(q3L)*((55491554575214198102159220722265*sin(q2L))/162259276829213363391578010288128 + cos(q2L)*((5557241208790345*cos(q1L))/9007199254740992 - (6384186990310915*sin(q1L))/9007199254740992) + (7514214926474921*sin(q2L)*((6384186990310915*cos(q1L))/9007199254740992 + (5557241208790345*sin(q1L))/9007199254740992))/36893488147419103232) + (9007199067919185*sin(q3L)*((57503643108550260546605243404275*cos(q1L))/81129638414606681695789005144064 + (50055177836018480443110068268825*sin(q1L))/81129638414606681695789005144064 - 46293577452674263141823442369649/664613997892457936451903530140172288))/9007199254740992))/36893488147419103232 - ((7514214926474921*cos(q4L))/36893488147419103232 + (4503599440548691*sin(q4L))/4503599627370496)*((7514214926474921*cos(q3L)*((55491554575214198102159220722265*cos(q2L))/162259276829213363391578010288128 + (7514214926474921*cos(q2L)*((6384186990310915*cos(q1L))/9007199254740992 + (5557241208790345*sin(q1L))/9007199254740992))/36893488147419103232 - sin(q2L)*((5557241208790345*cos(q1L))/9007199254740992 - (6384186990310915*sin(q1L))/9007199254740992)))/36893488147419103232 + (9007199067919185*cos(q3L)*((57503643108550260546605243404275*cos(q1L))/81129638414606681695789005144064 + (50055177836018480443110068268825*sin(q1L))/81129638414606681695789005144064 - 46293577452674263141823442369649/664613997892457936451903530140172288))/9007199254740992 + sin(q3L)*((55491554575214198102159220722265*sin(q2L))/162259276829213363391578010288128 + cos(q2L)*((5557241208790345*cos(q1L))/9007199254740992 - (6384186990310915*sin(q1L))/9007199254740992) + (7514214926474921*sin(q2L)*((6384186990310915*cos(q1L))/9007199254740992 + (5557241208790345*sin(q1L))/9007199254740992))/36893488147419103232))) + (7514214926474921*sin(q5L)*((7514214926474921*cos(q4L)*((7514214926474921*sin(q3L)*((55491554575214198102159220722265*cos(q2L))/162259276829213363391578010288128 + (7514214926474921*cos(q2L)*((6384186990310915*cos(q1L))/9007199254740992 + (5557241208790345*sin(q1L))/9007199254740992))/36893488147419103232 - sin(q2L)*((5557241208790345*cos(q1L))/9007199254740992 - (6384186990310915*sin(q1L))/9007199254740992)))/36893488147419103232 - cos(q3L)*((55491554575214198102159220722265*sin(q2L))/162259276829213363391578010288128 + cos(q2L)*((5557241208790345*cos(q1L))/9007199254740992 - (6384186990310915*sin(q1L))/9007199254740992) + (7514214926474921*sin(q2L)*((6384186990310915*cos(q1L))/9007199254740992 + (5557241208790345*sin(q1L))/9007199254740992))/36893488147419103232) + (9007199067919185*sin(q3L)*((57503643108550260546605243404275*cos(q1L))/81129638414606681695789005144064 + (50055177836018480443110068268825*sin(q1L))/81129638414606681695789005144064 - 46293577452674263141823442369649/664613997892457936451903530140172288))/9007199254740992))/36893488147419103232 - ((4503599440548691*cos(q4L))/4503599627370496 - (7514214926474921*sin(q4L))/36893488147419103232)*((7514214926474921*cos(q3L)*((55491554575214198102159220722265*cos(q2L))/162259276829213363391578010288128 + (7514214926474921*cos(q2L)*((6384186990310915*cos(q1L))/9007199254740992 + (5557241208790345*sin(q1L))/9007199254740992))/36893488147419103232 - sin(q2L)*((5557241208790345*cos(q1L))/9007199254740992 - (6384186990310915*sin(q1L))/9007199254740992)))/36893488147419103232 + (9007199067919185*cos(q3L)*((57503643108550260546605243404275*cos(q1L))/81129638414606681695789005144064 + (50055177836018480443110068268825*sin(q1L))/81129638414606681695789005144064 - 46293577452674263141823442369649/664613997892457936451903530140172288))/9007199254740992 + sin(q3L)*((55491554575214198102159220722265*sin(q2L))/162259276829213363391578010288128 + cos(q2L)*((5557241208790345*cos(q1L))/9007199254740992 - (6384186990310915*sin(q1L))/9007199254740992) + (7514214926474921*sin(q2L)*((6384186990310915*cos(q1L))/9007199254740992 + (5557241208790345*sin(q1L))/9007199254740992))/36893488147419103232))))/36893488147419103232))/9007199254740992000 + (83301539375654672537075965313343183841442266989297270401707771044036658496661398777306991*sin(q3L)*((57503643108550260546605243404275*cos(q1L))/81129638414606681695789005144064 + (50055177836018480443110068268825*sin(q1L))/81129638414606681695789005144064 - 46293577452674263141823442369649/664613997892457936451903530140172288))/4074071952668972172536891376818756322102936787331872501272280898708762599526673412366794752000 + (94754841554645069948206780163139*sin(q5L)*((7514214926474921*sin(q4L)*((7514214926474921*sin(q3L)*((55491554575214198102159220722265*cos(q2L))/162259276829213363391578010288128 + (7514214926474921*cos(q2L)*((6384186990310915*cos(q1L))/9007199254740992 + (5557241208790345*sin(q1L))/9007199254740992))/36893488147419103232 - sin(q2L)*((5557241208790345*cos(q1L))/9007199254740992 - (6384186990310915*sin(q1L))/9007199254740992)))/36893488147419103232 - cos(q3L)*((55491554575214198102159220722265*sin(q2L))/162259276829213363391578010288128 + cos(q2L)*((5557241208790345*cos(q1L))/9007199254740992 - (6384186990310915*sin(q1L))/9007199254740992) + (7514214926474921*sin(q2L)*((6384186990310915*cos(q1L))/9007199254740992 + (5557241208790345*sin(q1L))/9007199254740992))/36893488147419103232) + (9007199067919185*sin(q3L)*((57503643108550260546605243404275*cos(q1L))/81129638414606681695789005144064 + (50055177836018480443110068268825*sin(q1L))/81129638414606681695789005144064 - 46293577452674263141823442369649/664613997892457936451903530140172288))/9007199254740992))/36893488147419103232 - ((7514214926474921*cos(q4L))/36893488147419103232 + (4503599440548691*sin(q4L))/4503599627370496)*((7514214926474921*cos(q3L)*((55491554575214198102159220722265*cos(q2L))/162259276829213363391578010288128 + (7514214926474921*cos(q2L)*((6384186990310915*cos(q1L))/9007199254740992 + (5557241208790345*sin(q1L))/9007199254740992))/36893488147419103232 - sin(q2L)*((5557241208790345*cos(q1L))/9007199254740992 - (6384186990310915*sin(q1L))/9007199254740992)))/36893488147419103232 + (9007199067919185*cos(q3L)*((57503643108550260546605243404275*cos(q1L))/81129638414606681695789005144064 + (50055177836018480443110068268825*sin(q1L))/81129638414606681695789005144064 - 46293577452674263141823442369649/664613997892457936451903530140172288))/9007199254740992 + sin(q3L)*((55491554575214198102159220722265*sin(q2L))/162259276829213363391578010288128 + cos(q2L)*((5557241208790345*cos(q1L))/9007199254740992 - (6384186990310915*sin(q1L))/9007199254740992) + (7514214926474921*sin(q2L)*((6384186990310915*cos(q1L))/9007199254740992 + (5557241208790345*sin(q1L))/9007199254740992))/36893488147419103232))))/66461399789245793645190353014017228800 + (584133382113593486367040631332731*cos(q6L)*((9007199067919185*((4503599440548691*cos(q4L))/4503599627370496 - (7514214926474921*sin(q4L))/36893488147419103232)*((7514214926474921*cos(q3L)*((55491554575214198102159220722265*cos(q2L))/162259276829213363391578010288128 + (7514214926474921*cos(q2L)*((6384186990310915*cos(q1L))/9007199254740992 + (5557241208790345*sin(q1L))/9007199254740992))/36893488147419103232 - sin(q2L)*((5557241208790345*cos(q1L))/9007199254740992 - (6384186990310915*sin(q1L))/9007199254740992)))/36893488147419103232 + (9007199067919185*cos(q3L)*((57503643108550260546605243404275*cos(q1L))/81129638414606681695789005144064 + (50055177836018480443110068268825*sin(q1L))/81129638414606681695789005144064 - 46293577452674263141823442369649/664613997892457936451903530140172288))/9007199254740992 + sin(q3L)*((55491554575214198102159220722265*sin(q2L))/162259276829213363391578010288128 + cos(q2L)*((5557241208790345*cos(q1L))/9007199254740992 - (6384186990310915*sin(q1L))/9007199254740992) + (7514214926474921*sin(q2L)*((6384186990310915*cos(q1L))/9007199254740992 + (5557241208790345*sin(q1L))/9007199254740992))/36893488147419103232)))/9007199254740992 - (67682029681889335677290557259385*cos(q4L)*((7514214926474921*sin(q3L)*((55491554575214198102159220722265*cos(q2L))/162259276829213363391578010288128 + (7514214926474921*cos(q2L)*((6384186990310915*cos(q1L))/9007199254740992 + (5557241208790345*sin(q1L))/9007199254740992))/36893488147419103232 - sin(q2L)*((5557241208790345*cos(q1L))/9007199254740992 - (6384186990310915*sin(q1L))/9007199254740992)))/36893488147419103232 - cos(q3L)*((55491554575214198102159220722265*sin(q2L))/162259276829213363391578010288128 + cos(q2L)*((5557241208790345*cos(q1L))/9007199254740992 - (6384186990310915*sin(q1L))/9007199254740992) + (7514214926474921*sin(q2L)*((6384186990310915*cos(q1L))/9007199254740992 + (5557241208790345*sin(q1L))/9007199254740992))/36893488147419103232) + (9007199067919185*sin(q3L)*((57503643108550260546605243404275*cos(q1L))/81129638414606681695789005144064 + (50055177836018480443110068268825*sin(q1L))/81129638414606681695789005144064 - 46293577452674263141823442369649/664613997892457936451903530140172288))/9007199254740992))/332306998946228968225951765070086144 + (13258697167433729449897784796786197386719169465*cos(q3L)*((55491554575214198102159220722265*cos(q2L))/162259276829213363391578010288128 + (7514214926474921*cos(q2L)*((6384186990310915*cos(q1L))/9007199254740992 + (5557241208790345*sin(q1L))/9007199254740992))/36893488147419103232 - sin(q2L)*((5557241208790345*cos(q1L))/9007199254740992 - (6384186990310915*sin(q1L))/9007199254740992)))/1569275433846670190958947355801916604025588861116008628224 - (67682029681889335677290557259385*cos(q3L)*((55491554575214198102159220722265*sin(q2L))/162259276829213363391578010288128 + cos(q2L)*((5557241208790345*cos(q1L))/9007199254740992 - (6384186990310915*sin(q1L))/9007199254740992) + (7514214926474921*sin(q2L)*((6384186990310915*cos(q1L))/9007199254740992 + (5557241208790345*sin(q1L))/9007199254740992))/36893488147419103232))/332306998946228968225951765070086144 + (508577317689771495245073589786522929324694383585*sin(q3L)*((55491554575214198102159220722265*cos(q2L))/162259276829213363391578010288128 + (7514214926474921*cos(q2L)*((6384186990310915*cos(q1L))/9007199254740992 + (5557241208790345*sin(q1L))/9007199254740992))/36893488147419103232 - sin(q2L)*((5557241208790345*cos(q1L))/9007199254740992 - (6384186990310915*sin(q1L))/9007199254740992)))/12259964326927110866866776217202473468949912977468817408 + (15893040848161638993908057577265778144967053025*cos(q3L)*((57503643108550260546605243404275*cos(q1L))/81129638414606681695789005144064 + (50055177836018480443110068268825*sin(q1L))/81129638414606681695789005144064 - 46293577452674263141823442369649/664613997892457936451903530140172288))/383123885216472214589586756787577295904684780545900544 + (1764482024691522628700660907665*sin(q3L)*((55491554575214198102159220722265*sin(q2L))/162259276829213363391578010288128 + cos(q2L)*((5557241208790345*cos(q1L))/9007199254740992 - (6384186990310915*sin(q1L))/9007199254740992) + (7514214926474921*sin(q2L)*((6384186990310915*cos(q1L))/9007199254740992 + (5557241208790345*sin(q1L))/9007199254740992))/36893488147419103232))/42535295865117307932921825928971026432 + (609625514665592237562888769449172969868262801225*sin(q3L)*((57503643108550260546605243404275*cos(q1L))/81129638414606681695789005144064 + (50055177836018480443110068268825*sin(q1L))/81129638414606681695789005144064 - 46293577452674263141823442369649/664613997892457936451903530140172288))/2993155353253689176481146537402947624255349848014848))/16225927682921336339157801028812800, (608651409044468601*cos(q4L)*((7514214926474921*cos(q3L)*((55491554575214198102159220722265*cos(q2L))/162259276829213363391578010288128 + (7514214926474921*cos(q2L)*((6384186990310915*cos(q1L))/9007199254740992 + (5557241208790345*sin(q1L))/9007199254740992))/36893488147419103232 - sin(q2L)*((5557241208790345*cos(q1L))/9007199254740992 - (6384186990310915*sin(q1L))/9007199254740992)))/36893488147419103232 + (9007199067919185*cos(q3L)*((57503643108550260546605243404275*cos(q1L))/81129638414606681695789005144064 + (50055177836018480443110068268825*sin(q1L))/81129638414606681695789005144064 - 46293577452674263141823442369649/664613997892457936451903530140172288))/9007199254740992 + sin(q3L)*((55491554575214198102159220722265*sin(q2L))/162259276829213363391578010288128 + cos(q2L)*((5557241208790345*cos(q1L))/9007199254740992 - (6384186990310915*sin(q1L))/9007199254740992) + (7514214926474921*sin(q2L)*((6384186990310915*cos(q1L))/9007199254740992 + (5557241208790345*sin(q1L))/9007199254740992))/36893488147419103232)))/73786976294838206464000 - (610321541873521657855151997354401418608858870661075444886782706002880706727*sin(q4L)*((7514214926474921*cos(q3L)*((55491554575214198102159220722265*cos(q2L))/162259276829213363391578010288128 + (7514214926474921*cos(q2L)*((6384186990310915*cos(q1L))/9007199254740992 + (5557241208790345*sin(q1L))/9007199254740992))/36893488147419103232 - sin(q2L)*((5557241208790345*cos(q1L))/9007199254740992 - (6384186990310915*sin(q1L))/9007199254740992)))/36893488147419103232 + (9007199067919185*cos(q3L)*((57503643108550260546605243404275*cos(q1L))/81129638414606681695789005144064 + (50055177836018480443110068268825*sin(q1L))/81129638414606681695789005144064 - 46293577452674263141823442369649/664613997892457936451903530140172288))/9007199254740992 + sin(q3L)*((55491554575214198102159220722265*sin(q2L))/162259276829213363391578010288128 + cos(q2L)*((5557241208790345*cos(q1L))/9007199254740992 - (6384186990310915*sin(q1L))/9007199254740992) + (7514214926474921*sin(q2L)*((6384186990310915*cos(q1L))/9007199254740992 + (5557241208790345*sin(q1L))/9007199254740992))/36893488147419103232)))/11307821214581659709333104004754678501295896940003961331978279688272766566400000 - (584133382113593486367040631332731*cos(q6L)*((67682029681889335677290557259385*sin(q4L)*((7514214926474921*cos(q3L)*((55491554575214198102159220722265*cos(q2L))/162259276829213363391578010288128 + (7514214926474921*cos(q2L)*((6384186990310915*cos(q1L))/9007199254740992 + (5557241208790345*sin(q1L))/9007199254740992))/36893488147419103232 - sin(q2L)*((5557241208790345*cos(q1L))/9007199254740992 - (6384186990310915*sin(q1L))/9007199254740992)))/36893488147419103232 + (9007199067919185*cos(q3L)*((57503643108550260546605243404275*cos(q1L))/81129638414606681695789005144064 + (50055177836018480443110068268825*sin(q1L))/81129638414606681695789005144064 - 46293577452674263141823442369649/664613997892457936451903530140172288))/9007199254740992 + sin(q3L)*((55491554575214198102159220722265*sin(q2L))/162259276829213363391578010288128 + cos(q2L)*((5557241208790345*cos(q1L))/9007199254740992 - (6384186990310915*sin(q1L))/9007199254740992) + (7514214926474921*sin(q2L)*((6384186990310915*cos(q1L))/9007199254740992 + (5557241208790345*sin(q1L))/9007199254740992))/36893488147419103232)))/332306998946228968225951765070086144 + (9007199067919185*((7514214926474921*cos(q4L))/36893488147419103232 + (4503599440548691*sin(q4L))/4503599627370496)*((7514214926474921*sin(q3L)*((55491554575214198102159220722265*cos(q2L))/162259276829213363391578010288128 + (7514214926474921*cos(q2L)*((6384186990310915*cos(q1L))/9007199254740992 + (5557241208790345*sin(q1L))/9007199254740992))/36893488147419103232 - sin(q2L)*((5557241208790345*cos(q1L))/9007199254740992 - (6384186990310915*sin(q1L))/9007199254740992)))/36893488147419103232 - cos(q3L)*((55491554575214198102159220722265*sin(q2L))/162259276829213363391578010288128 + cos(q2L)*((5557241208790345*cos(q1L))/9007199254740992 - (6384186990310915*sin(q1L))/9007199254740992) + (7514214926474921*sin(q2L)*((6384186990310915*cos(q1L))/9007199254740992 + (5557241208790345*sin(q1L))/9007199254740992))/36893488147419103232) + (9007199067919185*sin(q3L)*((57503643108550260546605243404275*cos(q1L))/81129638414606681695789005144064 + (50055177836018480443110068268825*sin(q1L))/81129638414606681695789005144064 - 46293577452674263141823442369649/664613997892457936451903530140172288))/9007199254740992))/9007199254740992 - (9007199067919185*((9007199067919185*cos(q4L))/9007199254740992 - (234819211581865*sin(q4L))/1152921504606846976)*((432094733372955093709245836907320566011451687275*cos(q1L))/2993155353253689176481146537402947624255349848014848 - (499823478647255911063139966257565597426350154025*cos(q2L))/1461501637330902918203684832716283019655932542976 + (376125364442766701270516501597006072214248637825*sin(q1L))/2993155353253689176481146537402947624255349848014848 - (67682029681889335677290557259385*cos(q2L)*((6384186990310915*cos(q1L))/9007199254740992 + (5557241208790345*sin(q1L))/9007199254740992))/332306998946228968225951765070086144 + (9007199067919185*sin(q2L)*((5557241208790345*cos(q1L))/9007199254740992 - (6384186990310915*sin(q1L))/9007199254740992))/9007199254740992 - 347859890694807798813742879236295256254610072729/24519928653854221733733552434404946937899825954937634816))/9007199254740992))/16225927682921336339157801028812800 + (27*cos(q6L)*(cos(q5L)*((7514214926474921*cos(q4L)*((7514214926474921*cos(q3L)*((55491554575214198102159220722265*cos(q2L))/162259276829213363391578010288128 + (7514214926474921*cos(q2L)*((6384186990310915*cos(q1L))/9007199254740992 + (5557241208790345*sin(q1L))/9007199254740992))/36893488147419103232 - sin(q2L)*((5557241208790345*cos(q1L))/9007199254740992 - (6384186990310915*sin(q1L))/9007199254740992)))/36893488147419103232 + (9007199067919185*cos(q3L)*((57503643108550260546605243404275*cos(q1L))/81129638414606681695789005144064 + (50055177836018480443110068268825*sin(q1L))/81129638414606681695789005144064 - 46293577452674263141823442369649/664613997892457936451903530140172288))/9007199254740992 + sin(q3L)*((55491554575214198102159220722265*sin(q2L))/162259276829213363391578010288128 + cos(q2L)*((5557241208790345*cos(q1L))/9007199254740992 - (6384186990310915*sin(q1L))/9007199254740992) + (7514214926474921*sin(q2L)*((6384186990310915*cos(q1L))/9007199254740992 + (5557241208790345*sin(q1L))/9007199254740992))/36893488147419103232)))/36893488147419103232 + ((4503599440548691*cos(q4L))/4503599627370496 - (7514214926474921*sin(q4L))/36893488147419103232)*((7514214926474921*sin(q3L)*((55491554575214198102159220722265*cos(q2L))/162259276829213363391578010288128 + (7514214926474921*cos(q2L)*((6384186990310915*cos(q1L))/9007199254740992 + (5557241208790345*sin(q1L))/9007199254740992))/36893488147419103232 - sin(q2L)*((5557241208790345*cos(q1L))/9007199254740992 - (6384186990310915*sin(q1L))/9007199254740992)))/36893488147419103232 - cos(q3L)*((55491554575214198102159220722265*sin(q2L))/162259276829213363391578010288128 + cos(q2L)*((5557241208790345*cos(q1L))/9007199254740992 - (6384186990310915*sin(q1L))/9007199254740992) + (7514214926474921*sin(q2L)*((6384186990310915*cos(q1L))/9007199254740992 + (5557241208790345*sin(q1L))/9007199254740992))/36893488147419103232) + (9007199067919185*sin(q3L)*((57503643108550260546605243404275*cos(q1L))/81129638414606681695789005144064 + (50055177836018480443110068268825*sin(q1L))/81129638414606681695789005144064 - 46293577452674263141823442369649/664613997892457936451903530140172288))/9007199254740992) + ((234819211581865*cos(q4L))/1152921504606846976 + (9007199067919185*sin(q4L))/9007199254740992)*((432094733372955093709245836907320566011451687275*cos(q1L))/2993155353253689176481146537402947624255349848014848 - (499823478647255911063139966257565597426350154025*cos(q2L))/1461501637330902918203684832716283019655932542976 + (376125364442766701270516501597006072214248637825*sin(q1L))/2993155353253689176481146537402947624255349848014848 - (67682029681889335677290557259385*cos(q2L)*((6384186990310915*cos(q1L))/9007199254740992 + (5557241208790345*sin(q1L))/9007199254740992))/332306998946228968225951765070086144 + (9007199067919185*sin(q2L)*((5557241208790345*cos(q1L))/9007199254740992 - (6384186990310915*sin(q1L))/9007199254740992))/9007199254740992 - 347859890694807798813742879236295256254610072729/24519928653854221733733552434404946937899825954937634816)) + (7514214926474921*sin(q5L)*((7514214926474921*sin(q4L)*((7514214926474921*cos(q3L)*((55491554575214198102159220722265*cos(q2L))/162259276829213363391578010288128 + (7514214926474921*cos(q2L)*((6384186990310915*cos(q1L))/9007199254740992 + (5557241208790345*sin(q1L))/9007199254740992))/36893488147419103232 - sin(q2L)*((5557241208790345*cos(q1L))/9007199254740992 - (6384186990310915*sin(q1L))/9007199254740992)))/36893488147419103232 + (9007199067919185*cos(q3L)*((57503643108550260546605243404275*cos(q1L))/81129638414606681695789005144064 + (50055177836018480443110068268825*sin(q1L))/81129638414606681695789005144064 - 46293577452674263141823442369649/664613997892457936451903530140172288))/9007199254740992 + sin(q3L)*((55491554575214198102159220722265*sin(q2L))/162259276829213363391578010288128 + cos(q2L)*((5557241208790345*cos(q1L))/9007199254740992 - (6384186990310915*sin(q1L))/9007199254740992) + (7514214926474921*sin(q2L)*((6384186990310915*cos(q1L))/9007199254740992 + (5557241208790345*sin(q1L))/9007199254740992))/36893488147419103232)))/36893488147419103232 + ((7514214926474921*cos(q4L))/36893488147419103232 + (4503599440548691*sin(q4L))/4503599627370496)*((7514214926474921*sin(q3L)*((55491554575214198102159220722265*cos(q2L))/162259276829213363391578010288128 + (7514214926474921*cos(q2L)*((6384186990310915*cos(q1L))/9007199254740992 + (5557241208790345*sin(q1L))/9007199254740992))/36893488147419103232 - sin(q2L)*((5557241208790345*cos(q1L))/9007199254740992 - (6384186990310915*sin(q1L))/9007199254740992)))/36893488147419103232 - cos(q3L)*((55491554575214198102159220722265*sin(q2L))/162259276829213363391578010288128 + cos(q2L)*((5557241208790345*cos(q1L))/9007199254740992 - (6384186990310915*sin(q1L))/9007199254740992) + (7514214926474921*sin(q2L)*((6384186990310915*cos(q1L))/9007199254740992 + (5557241208790345*sin(q1L))/9007199254740992))/36893488147419103232) + (9007199067919185*sin(q3L)*((57503643108550260546605243404275*cos(q1L))/81129638414606681695789005144064 + (50055177836018480443110068268825*sin(q1L))/81129638414606681695789005144064 - 46293577452674263141823442369649/664613997892457936451903530140172288))/9007199254740992) - ((9007199067919185*cos(q4L))/9007199254740992 - (234819211581865*sin(q4L))/1152921504606846976)*((432094733372955093709245836907320566011451687275*cos(q1L))/2993155353253689176481146537402947624255349848014848 - (499823478647255911063139966257565597426350154025*cos(q2L))/1461501637330902918203684832716283019655932542976 + (376125364442766701270516501597006072214248637825*sin(q1L))/2993155353253689176481146537402947624255349848014848 - (67682029681889335677290557259385*cos(q2L)*((6384186990310915*cos(q1L))/9007199254740992 + (5557241208790345*sin(q1L))/9007199254740992))/332306998946228968225951765070086144 + (9007199067919185*sin(q2L)*((5557241208790345*cos(q1L))/9007199254740992 - (6384186990310915*sin(q1L))/9007199254740992))/9007199254740992 - 347859890694807798813742879236295256254610072729/24519928653854221733733552434404946937899825954937634816)))/36893488147419103232))/1000 + (2436553109258773196144549622003023*cos(q6L)*(sin(q5L)*((7514214926474921*cos(q4L)*((7514214926474921*cos(q3L)*((55491554575214198102159220722265*cos(q2L))/162259276829213363391578010288128 + (7514214926474921*cos(q2L)*((6384186990310915*cos(q1L))/9007199254740992 + (5557241208790345*sin(q1L))/9007199254740992))/36893488147419103232 - sin(q2L)*((5557241208790345*cos(q1L))/9007199254740992 - (6384186990310915*sin(q1L))/9007199254740992)))/36893488147419103232 + (9007199067919185*cos(q3L)*((57503643108550260546605243404275*cos(q1L))/81129638414606681695789005144064 + (50055177836018480443110068268825*sin(q1L))/81129638414606681695789005144064 - 46293577452674263141823442369649/664613997892457936451903530140172288))/9007199254740992 + sin(q3L)*((55491554575214198102159220722265*sin(q2L))/162259276829213363391578010288128 + cos(q2L)*((5557241208790345*cos(q1L))/9007199254740992 - (6384186990310915*sin(q1L))/9007199254740992) + (7514214926474921*sin(q2L)*((6384186990310915*cos(q1L))/9007199254740992 + (5557241208790345*sin(q1L))/9007199254740992))/36893488147419103232)))/36893488147419103232 + ((4503599440548691*cos(q4L))/4503599627370496 - (7514214926474921*sin(q4L))/36893488147419103232)*((7514214926474921*sin(q3L)*((55491554575214198102159220722265*cos(q2L))/162259276829213363391578010288128 + (7514214926474921*cos(q2L)*((6384186990310915*cos(q1L))/9007199254740992 + (5557241208790345*sin(q1L))/9007199254740992))/36893488147419103232 - sin(q2L)*((5557241208790345*cos(q1L))/9007199254740992 - (6384186990310915*sin(q1L))/9007199254740992)))/36893488147419103232 - cos(q3L)*((55491554575214198102159220722265*sin(q2L))/162259276829213363391578010288128 + cos(q2L)*((5557241208790345*cos(q1L))/9007199254740992 - (6384186990310915*sin(q1L))/9007199254740992) + (7514214926474921*sin(q2L)*((6384186990310915*cos(q1L))/9007199254740992 + (5557241208790345*sin(q1L))/9007199254740992))/36893488147419103232) + (9007199067919185*sin(q3L)*((57503643108550260546605243404275*cos(q1L))/81129638414606681695789005144064 + (50055177836018480443110068268825*sin(q1L))/81129638414606681695789005144064 - 46293577452674263141823442369649/664613997892457936451903530140172288))/9007199254740992) + ((234819211581865*cos(q4L))/1152921504606846976 + (9007199067919185*sin(q4L))/9007199254740992)*((432094733372955093709245836907320566011451687275*cos(q1L))/2993155353253689176481146537402947624255349848014848 - (499823478647255911063139966257565597426350154025*cos(q2L))/1461501637330902918203684832716283019655932542976 + (376125364442766701270516501597006072214248637825*sin(q1L))/2993155353253689176481146537402947624255349848014848 - (67682029681889335677290557259385*cos(q2L)*((6384186990310915*cos(q1L))/9007199254740992 + (5557241208790345*sin(q1L))/9007199254740992))/332306998946228968225951765070086144 + (9007199067919185*sin(q2L)*((5557241208790345*cos(q1L))/9007199254740992 - (6384186990310915*sin(q1L))/9007199254740992))/9007199254740992 - 347859890694807798813742879236295256254610072729/24519928653854221733733552434404946937899825954937634816)) - (7514214926474921*cos(q5L)*((7514214926474921*sin(q4L)*((7514214926474921*cos(q3L)*((55491554575214198102159220722265*cos(q2L))/162259276829213363391578010288128 + (7514214926474921*cos(q2L)*((6384186990310915*cos(q1L))/9007199254740992 + (5557241208790345*sin(q1L))/9007199254740992))/36893488147419103232 - sin(q2L)*((5557241208790345*cos(q1L))/9007199254740992 - (6384186990310915*sin(q1L))/9007199254740992)))/36893488147419103232 + (9007199067919185*cos(q3L)*((57503643108550260546605243404275*cos(q1L))/81129638414606681695789005144064 + (50055177836018480443110068268825*sin(q1L))/81129638414606681695789005144064 - 46293577452674263141823442369649/664613997892457936451903530140172288))/9007199254740992 + sin(q3L)*((55491554575214198102159220722265*sin(q2L))/162259276829213363391578010288128 + cos(q2L)*((5557241208790345*cos(q1L))/9007199254740992 - (6384186990310915*sin(q1L))/9007199254740992) + (7514214926474921*sin(q2L)*((6384186990310915*cos(q1L))/9007199254740992 + (5557241208790345*sin(q1L))/9007199254740992))/36893488147419103232)))/36893488147419103232 + ((7514214926474921*cos(q4L))/36893488147419103232 + (4503599440548691*sin(q4L))/4503599627370496)*((7514214926474921*sin(q3L)*((55491554575214198102159220722265*cos(q2L))/162259276829213363391578010288128 + (7514214926474921*cos(q2L)*((6384186990310915*cos(q1L))/9007199254740992 + (5557241208790345*sin(q1L))/9007199254740992))/36893488147419103232 - sin(q2L)*((5557241208790345*cos(q1L))/9007199254740992 - (6384186990310915*sin(q1L))/9007199254740992)))/36893488147419103232 - cos(q3L)*((55491554575214198102159220722265*sin(q2L))/162259276829213363391578010288128 + cos(q2L)*((5557241208790345*cos(q1L))/9007199254740992 - (6384186990310915*sin(q1L))/9007199254740992) + (7514214926474921*sin(q2L)*((6384186990310915*cos(q1L))/9007199254740992 + (5557241208790345*sin(q1L))/9007199254740992))/36893488147419103232) + (9007199067919185*sin(q3L)*((57503643108550260546605243404275*cos(q1L))/81129638414606681695789005144064 + (50055177836018480443110068268825*sin(q1L))/81129638414606681695789005144064 - 46293577452674263141823442369649/664613997892457936451903530140172288))/9007199254740992) - ((9007199067919185*cos(q4L))/9007199254740992 - (234819211581865*sin(q4L))/1152921504606846976)*((432094733372955093709245836907320566011451687275*cos(q1L))/2993155353253689176481146537402947624255349848014848 - (499823478647255911063139966257565597426350154025*cos(q2L))/1461501637330902918203684832716283019655932542976 + (376125364442766701270516501597006072214248637825*sin(q1L))/2993155353253689176481146537402947624255349848014848 - (67682029681889335677290557259385*cos(q2L)*((6384186990310915*cos(q1L))/9007199254740992 + (5557241208790345*sin(q1L))/9007199254740992))/332306998946228968225951765070086144 + (9007199067919185*sin(q2L)*((5557241208790345*cos(q1L))/9007199254740992 - (6384186990310915*sin(q1L))/9007199254740992))/9007199254740992 - 347859890694807798813742879236295256254610072729/24519928653854221733733552434404946937899825954937634816)))/36893488147419103232))/332306998946228968225951765070086144000 - (48638874966763599*sin(q6L)*((67682029681889335677290557259385*sin(q4L)*((7514214926474921*cos(q3L)*((55491554575214198102159220722265*cos(q2L))/162259276829213363391578010288128 + (7514214926474921*cos(q2L)*((6384186990310915*cos(q1L))/9007199254740992 + (5557241208790345*sin(q1L))/9007199254740992))/36893488147419103232 - sin(q2L)*((5557241208790345*cos(q1L))/9007199254740992 - (6384186990310915*sin(q1L))/9007199254740992)))/36893488147419103232 + (9007199067919185*cos(q3L)*((57503643108550260546605243404275*cos(q1L))/81129638414606681695789005144064 + (50055177836018480443110068268825*sin(q1L))/81129638414606681695789005144064 - 46293577452674263141823442369649/664613997892457936451903530140172288))/9007199254740992 + sin(q3L)*((55491554575214198102159220722265*sin(q2L))/162259276829213363391578010288128 + cos(q2L)*((5557241208790345*cos(q1L))/9007199254740992 - (6384186990310915*sin(q1L))/9007199254740992) + (7514214926474921*sin(q2L)*((6384186990310915*cos(q1L))/9007199254740992 + (5557241208790345*sin(q1L))/9007199254740992))/36893488147419103232)))/332306998946228968225951765070086144 + (9007199067919185*((7514214926474921*cos(q4L))/36893488147419103232 + (4503599440548691*sin(q4L))/4503599627370496)*((7514214926474921*sin(q3L)*((55491554575214198102159220722265*cos(q2L))/162259276829213363391578010288128 + (7514214926474921*cos(q2L)*((6384186990310915*cos(q1L))/9007199254740992 + (5557241208790345*sin(q1L))/9007199254740992))/36893488147419103232 - sin(q2L)*((5557241208790345*cos(q1L))/9007199254740992 - (6384186990310915*sin(q1L))/9007199254740992)))/36893488147419103232 - cos(q3L)*((55491554575214198102159220722265*sin(q2L))/162259276829213363391578010288128 + cos(q2L)*((5557241208790345*cos(q1L))/9007199254740992 - (6384186990310915*sin(q1L))/9007199254740992) + (7514214926474921*sin(q2L)*((6384186990310915*cos(q1L))/9007199254740992 + (5557241208790345*sin(q1L))/9007199254740992))/36893488147419103232) + (9007199067919185*sin(q3L)*((57503643108550260546605243404275*cos(q1L))/81129638414606681695789005144064 + (50055177836018480443110068268825*sin(q1L))/81129638414606681695789005144064 - 46293577452674263141823442369649/664613997892457936451903530140172288))/9007199254740992))/9007199254740992 - (9007199067919185*((9007199067919185*cos(q4L))/9007199254740992 - (234819211581865*sin(q4L))/1152921504606846976)*((432094733372955093709245836907320566011451687275*cos(q1L))/2993155353253689176481146537402947624255349848014848 - (499823478647255911063139966257565597426350154025*cos(q2L))/1461501637330902918203684832716283019655932542976 + (376125364442766701270516501597006072214248637825*sin(q1L))/2993155353253689176481146537402947624255349848014848 - (67682029681889335677290557259385*cos(q2L)*((6384186990310915*cos(q1L))/9007199254740992 + (5557241208790345*sin(q1L))/9007199254740992))/332306998946228968225951765070086144 + (9007199067919185*sin(q2L)*((5557241208790345*cos(q1L))/9007199254740992 - (6384186990310915*sin(q1L))/9007199254740992))/9007199254740992 - 347859890694807798813742879236295256254610072729/24519928653854221733733552434404946937899825954937634816))/9007199254740992))/1801439850948198400 - (324259171862923063*sin(q6L)*(cos(q5L)*((7514214926474921*cos(q4L)*((7514214926474921*cos(q3L)*((55491554575214198102159220722265*cos(q2L))/162259276829213363391578010288128 + (7514214926474921*cos(q2L)*((6384186990310915*cos(q1L))/9007199254740992 + (5557241208790345*sin(q1L))/9007199254740992))/36893488147419103232 - sin(q2L)*((5557241208790345*cos(q1L))/9007199254740992 - (6384186990310915*sin(q1L))/9007199254740992)))/36893488147419103232 + (9007199067919185*cos(q3L)*((57503643108550260546605243404275*cos(q1L))/81129638414606681695789005144064 + (50055177836018480443110068268825*sin(q1L))/81129638414606681695789005144064 - 46293577452674263141823442369649/664613997892457936451903530140172288))/9007199254740992 + sin(q3L)*((55491554575214198102159220722265*sin(q2L))/162259276829213363391578010288128 + cos(q2L)*((5557241208790345*cos(q1L))/9007199254740992 - (6384186990310915*sin(q1L))/9007199254740992) + (7514214926474921*sin(q2L)*((6384186990310915*cos(q1L))/9007199254740992 + (5557241208790345*sin(q1L))/9007199254740992))/36893488147419103232)))/36893488147419103232 + ((4503599440548691*cos(q4L))/4503599627370496 - (7514214926474921*sin(q4L))/36893488147419103232)*((7514214926474921*sin(q3L)*((55491554575214198102159220722265*cos(q2L))/162259276829213363391578010288128 + (7514214926474921*cos(q2L)*((6384186990310915*cos(q1L))/9007199254740992 + (5557241208790345*sin(q1L))/9007199254740992))/36893488147419103232 - sin(q2L)*((5557241208790345*cos(q1L))/9007199254740992 - (6384186990310915*sin(q1L))/9007199254740992)))/36893488147419103232 - cos(q3L)*((55491554575214198102159220722265*sin(q2L))/162259276829213363391578010288128 + cos(q2L)*((5557241208790345*cos(q1L))/9007199254740992 - (6384186990310915*sin(q1L))/9007199254740992) + (7514214926474921*sin(q2L)*((6384186990310915*cos(q1L))/9007199254740992 + (5557241208790345*sin(q1L))/9007199254740992))/36893488147419103232) + (9007199067919185*sin(q3L)*((57503643108550260546605243404275*cos(q1L))/81129638414606681695789005144064 + (50055177836018480443110068268825*sin(q1L))/81129638414606681695789005144064 - 46293577452674263141823442369649/664613997892457936451903530140172288))/9007199254740992) + ((234819211581865*cos(q4L))/1152921504606846976 + (9007199067919185*sin(q4L))/9007199254740992)*((432094733372955093709245836907320566011451687275*cos(q1L))/2993155353253689176481146537402947624255349848014848 - (499823478647255911063139966257565597426350154025*cos(q2L))/1461501637330902918203684832716283019655932542976 + (376125364442766701270516501597006072214248637825*sin(q1L))/2993155353253689176481146537402947624255349848014848 - (67682029681889335677290557259385*cos(q2L)*((6384186990310915*cos(q1L))/9007199254740992 + (5557241208790345*sin(q1L))/9007199254740992))/332306998946228968225951765070086144 + (9007199067919185*sin(q2L)*((5557241208790345*cos(q1L))/9007199254740992 - (6384186990310915*sin(q1L))/9007199254740992))/9007199254740992 - 347859890694807798813742879236295256254610072729/24519928653854221733733552434404946937899825954937634816)) + (7514214926474921*sin(q5L)*((7514214926474921*sin(q4L)*((7514214926474921*cos(q3L)*((55491554575214198102159220722265*cos(q2L))/162259276829213363391578010288128 + (7514214926474921*cos(q2L)*((6384186990310915*cos(q1L))/9007199254740992 + (5557241208790345*sin(q1L))/9007199254740992))/36893488147419103232 - sin(q2L)*((5557241208790345*cos(q1L))/9007199254740992 - (6384186990310915*sin(q1L))/9007199254740992)))/36893488147419103232 + (9007199067919185*cos(q3L)*((57503643108550260546605243404275*cos(q1L))/81129638414606681695789005144064 + (50055177836018480443110068268825*sin(q1L))/81129638414606681695789005144064 - 46293577452674263141823442369649/664613997892457936451903530140172288))/9007199254740992 + sin(q3L)*((55491554575214198102159220722265*sin(q2L))/162259276829213363391578010288128 + cos(q2L)*((5557241208790345*cos(q1L))/9007199254740992 - (6384186990310915*sin(q1L))/9007199254740992) + (7514214926474921*sin(q2L)*((6384186990310915*cos(q1L))/9007199254740992 + (5557241208790345*sin(q1L))/9007199254740992))/36893488147419103232)))/36893488147419103232 + ((7514214926474921*cos(q4L))/36893488147419103232 + (4503599440548691*sin(q4L))/4503599627370496)*((7514214926474921*sin(q3L)*((55491554575214198102159220722265*cos(q2L))/162259276829213363391578010288128 + (7514214926474921*cos(q2L)*((6384186990310915*cos(q1L))/9007199254740992 + (5557241208790345*sin(q1L))/9007199254740992))/36893488147419103232 - sin(q2L)*((5557241208790345*cos(q1L))/9007199254740992 - (6384186990310915*sin(q1L))/9007199254740992)))/36893488147419103232 - cos(q3L)*((55491554575214198102159220722265*sin(q2L))/162259276829213363391578010288128 + cos(q2L)*((5557241208790345*cos(q1L))/9007199254740992 - (6384186990310915*sin(q1L))/9007199254740992) + (7514214926474921*sin(q2L)*((6384186990310915*cos(q1L))/9007199254740992 + (5557241208790345*sin(q1L))/9007199254740992))/36893488147419103232) + (9007199067919185*sin(q3L)*((57503643108550260546605243404275*cos(q1L))/81129638414606681695789005144064 + (50055177836018480443110068268825*sin(q1L))/81129638414606681695789005144064 - 46293577452674263141823442369649/664613997892457936451903530140172288))/9007199254740992) - ((9007199067919185*cos(q4L))/9007199254740992 - (234819211581865*sin(q4L))/1152921504606846976)*((432094733372955093709245836907320566011451687275*cos(q1L))/2993155353253689176481146537402947624255349848014848 - (499823478647255911063139966257565597426350154025*cos(q2L))/1461501637330902918203684832716283019655932542976 + (376125364442766701270516501597006072214248637825*sin(q1L))/2993155353253689176481146537402947624255349848014848 - (67682029681889335677290557259385*cos(q2L)*((6384186990310915*cos(q1L))/9007199254740992 + (5557241208790345*sin(q1L))/9007199254740992))/332306998946228968225951765070086144 + (9007199067919185*sin(q2L)*((5557241208790345*cos(q1L))/9007199254740992 - (6384186990310915*sin(q1L))/9007199254740992))/9007199254740992 - 347859890694807798813742879236295256254610072729/24519928653854221733733552434404946937899825954937634816)))/36893488147419103232))/9007199254740992000 + (202883803014822867*sin(q6L)*(sin(q5L)*((7514214926474921*cos(q4L)*((7514214926474921*cos(q3L)*((55491554575214198102159220722265*cos(q2L))/162259276829213363391578010288128 + (7514214926474921*cos(q2L)*((6384186990310915*cos(q1L))/9007199254740992 + (5557241208790345*sin(q1L))/9007199254740992))/36893488147419103232 - sin(q2L)*((5557241208790345*cos(q1L))/9007199254740992 - (6384186990310915*sin(q1L))/9007199254740992)))/36893488147419103232 + (9007199067919185*cos(q3L)*((57503643108550260546605243404275*cos(q1L))/81129638414606681695789005144064 + (50055177836018480443110068268825*sin(q1L))/81129638414606681695789005144064 - 46293577452674263141823442369649/664613997892457936451903530140172288))/9007199254740992 + sin(q3L)*((55491554575214198102159220722265*sin(q2L))/162259276829213363391578010288128 + cos(q2L)*((5557241208790345*cos(q1L))/9007199254740992 - (6384186990310915*sin(q1L))/9007199254740992) + (7514214926474921*sin(q2L)*((6384186990310915*cos(q1L))/9007199254740992 + (5557241208790345*sin(q1L))/9007199254740992))/36893488147419103232)))/36893488147419103232 + ((4503599440548691*cos(q4L))/4503599627370496 - (7514214926474921*sin(q4L))/36893488147419103232)*((7514214926474921*sin(q3L)*((55491554575214198102159220722265*cos(q2L))/162259276829213363391578010288128 + (7514214926474921*cos(q2L)*((6384186990310915*cos(q1L))/9007199254740992 + (5557241208790345*sin(q1L))/9007199254740992))/36893488147419103232 - sin(q2L)*((5557241208790345*cos(q1L))/9007199254740992 - (6384186990310915*sin(q1L))/9007199254740992)))/36893488147419103232 - cos(q3L)*((55491554575214198102159220722265*sin(q2L))/162259276829213363391578010288128 + cos(q2L)*((5557241208790345*cos(q1L))/9007199254740992 - (6384186990310915*sin(q1L))/9007199254740992) + (7514214926474921*sin(q2L)*((6384186990310915*cos(q1L))/9007199254740992 + (5557241208790345*sin(q1L))/9007199254740992))/36893488147419103232) + (9007199067919185*sin(q3L)*((57503643108550260546605243404275*cos(q1L))/81129638414606681695789005144064 + (50055177836018480443110068268825*sin(q1L))/81129638414606681695789005144064 - 46293577452674263141823442369649/664613997892457936451903530140172288))/9007199254740992) + ((234819211581865*cos(q4L))/1152921504606846976 + (9007199067919185*sin(q4L))/9007199254740992)*((432094733372955093709245836907320566011451687275*cos(q1L))/2993155353253689176481146537402947624255349848014848 - (499823478647255911063139966257565597426350154025*cos(q2L))/1461501637330902918203684832716283019655932542976 + (376125364442766701270516501597006072214248637825*sin(q1L))/2993155353253689176481146537402947624255349848014848 - (67682029681889335677290557259385*cos(q2L)*((6384186990310915*cos(q1L))/9007199254740992 + (5557241208790345*sin(q1L))/9007199254740992))/332306998946228968225951765070086144 + (9007199067919185*sin(q2L)*((5557241208790345*cos(q1L))/9007199254740992 - (6384186990310915*sin(q1L))/9007199254740992))/9007199254740992 - 347859890694807798813742879236295256254610072729/24519928653854221733733552434404946937899825954937634816)) - (7514214926474921*cos(q5L)*((7514214926474921*sin(q4L)*((7514214926474921*cos(q3L)*((55491554575214198102159220722265*cos(q2L))/162259276829213363391578010288128 + (7514214926474921*cos(q2L)*((6384186990310915*cos(q1L))/9007199254740992 + (5557241208790345*sin(q1L))/9007199254740992))/36893488147419103232 - sin(q2L)*((5557241208790345*cos(q1L))/9007199254740992 - (6384186990310915*sin(q1L))/9007199254740992)))/36893488147419103232 + (9007199067919185*cos(q3L)*((57503643108550260546605243404275*cos(q1L))/81129638414606681695789005144064 + (50055177836018480443110068268825*sin(q1L))/81129638414606681695789005144064 - 46293577452674263141823442369649/664613997892457936451903530140172288))/9007199254740992 + sin(q3L)*((55491554575214198102159220722265*sin(q2L))/162259276829213363391578010288128 + cos(q2L)*((5557241208790345*cos(q1L))/9007199254740992 - (6384186990310915*sin(q1L))/9007199254740992) + (7514214926474921*sin(q2L)*((6384186990310915*cos(q1L))/9007199254740992 + (5557241208790345*sin(q1L))/9007199254740992))/36893488147419103232)))/36893488147419103232 + ((7514214926474921*cos(q4L))/36893488147419103232 + (4503599440548691*sin(q4L))/4503599627370496)*((7514214926474921*sin(q3L)*((55491554575214198102159220722265*cos(q2L))/162259276829213363391578010288128 + (7514214926474921*cos(q2L)*((6384186990310915*cos(q1L))/9007199254740992 + (5557241208790345*sin(q1L))/9007199254740992))/36893488147419103232 - sin(q2L)*((5557241208790345*cos(q1L))/9007199254740992 - (6384186990310915*sin(q1L))/9007199254740992)))/36893488147419103232 - cos(q3L)*((55491554575214198102159220722265*sin(q2L))/162259276829213363391578010288128 + cos(q2L)*((5557241208790345*cos(q1L))/9007199254740992 - (6384186990310915*sin(q1L))/9007199254740992) + (7514214926474921*sin(q2L)*((6384186990310915*cos(q1L))/9007199254740992 + (5557241208790345*sin(q1L))/9007199254740992))/36893488147419103232) + (9007199067919185*sin(q3L)*((57503643108550260546605243404275*cos(q1L))/81129638414606681695789005144064 + (50055177836018480443110068268825*sin(q1L))/81129638414606681695789005144064 - 46293577452674263141823442369649/664613997892457936451903530140172288))/9007199254740992) - ((9007199067919185*cos(q4L))/9007199254740992 - (234819211581865*sin(q4L))/1152921504606846976)*((432094733372955093709245836907320566011451687275*cos(q1L))/2993155353253689176481146537402947624255349848014848 - (499823478647255911063139966257565597426350154025*cos(q2L))/1461501637330902918203684832716283019655932542976 + (376125364442766701270516501597006072214248637825*sin(q1L))/2993155353253689176481146537402947624255349848014848 - (67682029681889335677290557259385*cos(q2L)*((6384186990310915*cos(q1L))/9007199254740992 + (5557241208790345*sin(q1L))/9007199254740992))/332306998946228968225951765070086144 + (9007199067919185*sin(q2L)*((5557241208790345*cos(q1L))/9007199254740992 - (6384186990310915*sin(q1L))/9007199254740992))/9007199254740992 - 347859890694807798813742879236295256254610072729/24519928653854221733733552434404946937899825954937634816)))/36893488147419103232))/36893488147419103232000 - (27*cos(q5L)*((7514214926474921*cos(q4L)*((7514214926474921*cos(q3L)*((55491554575214198102159220722265*cos(q2L))/162259276829213363391578010288128 + (7514214926474921*cos(q2L)*((6384186990310915*cos(q1L))/9007199254740992 + (5557241208790345*sin(q1L))/9007199254740992))/36893488147419103232 - sin(q2L)*((5557241208790345*cos(q1L))/9007199254740992 - (6384186990310915*sin(q1L))/9007199254740992)))/36893488147419103232 + (9007199067919185*cos(q3L)*((57503643108550260546605243404275*cos(q1L))/81129638414606681695789005144064 + (50055177836018480443110068268825*sin(q1L))/81129638414606681695789005144064 - 46293577452674263141823442369649/664613997892457936451903530140172288))/9007199254740992 + sin(q3L)*((55491554575214198102159220722265*sin(q2L))/162259276829213363391578010288128 + cos(q2L)*((5557241208790345*cos(q1L))/9007199254740992 - (6384186990310915*sin(q1L))/9007199254740992) + (7514214926474921*sin(q2L)*((6384186990310915*cos(q1L))/9007199254740992 + (5557241208790345*sin(q1L))/9007199254740992))/36893488147419103232)))/36893488147419103232 + ((4503599440548691*cos(q4L))/4503599627370496 - (7514214926474921*sin(q4L))/36893488147419103232)*((7514214926474921*sin(q3L)*((55491554575214198102159220722265*cos(q2L))/162259276829213363391578010288128 + (7514214926474921*cos(q2L)*((6384186990310915*cos(q1L))/9007199254740992 + (5557241208790345*sin(q1L))/9007199254740992))/36893488147419103232 - sin(q2L)*((5557241208790345*cos(q1L))/9007199254740992 - (6384186990310915*sin(q1L))/9007199254740992)))/36893488147419103232 - cos(q3L)*((55491554575214198102159220722265*sin(q2L))/162259276829213363391578010288128 + cos(q2L)*((5557241208790345*cos(q1L))/9007199254740992 - (6384186990310915*sin(q1L))/9007199254740992) + (7514214926474921*sin(q2L)*((6384186990310915*cos(q1L))/9007199254740992 + (5557241208790345*sin(q1L))/9007199254740992))/36893488147419103232) + (9007199067919185*sin(q3L)*((57503643108550260546605243404275*cos(q1L))/81129638414606681695789005144064 + (50055177836018480443110068268825*sin(q1L))/81129638414606681695789005144064 - 46293577452674263141823442369649/664613997892457936451903530140172288))/9007199254740992) + ((234819211581865*cos(q4L))/1152921504606846976 + (9007199067919185*sin(q4L))/9007199254740992)*((432094733372955093709245836907320566011451687275*cos(q1L))/2993155353253689176481146537402947624255349848014848 - (499823478647255911063139966257565597426350154025*cos(q2L))/1461501637330902918203684832716283019655932542976 + (376125364442766701270516501597006072214248637825*sin(q1L))/2993155353253689176481146537402947624255349848014848 - (67682029681889335677290557259385*cos(q2L)*((6384186990310915*cos(q1L))/9007199254740992 + (5557241208790345*sin(q1L))/9007199254740992))/332306998946228968225951765070086144 + (9007199067919185*sin(q2L)*((5557241208790345*cos(q1L))/9007199254740992 - (6384186990310915*sin(q1L))/9007199254740992))/9007199254740992 - 347859890694807798813742879236295256254610072729/24519928653854221733733552434404946937899825954937634816)))/1000 - (94754841554645069948206780163139*sin(q5L)*((7514214926474921*cos(q4L)*((7514214926474921*cos(q3L)*((55491554575214198102159220722265*cos(q2L))/162259276829213363391578010288128 + (7514214926474921*cos(q2L)*((6384186990310915*cos(q1L))/9007199254740992 + (5557241208790345*sin(q1L))/9007199254740992))/36893488147419103232 - sin(q2L)*((5557241208790345*cos(q1L))/9007199254740992 - (6384186990310915*sin(q1L))/9007199254740992)))/36893488147419103232 + (9007199067919185*cos(q3L)*((57503643108550260546605243404275*cos(q1L))/81129638414606681695789005144064 + (50055177836018480443110068268825*sin(q1L))/81129638414606681695789005144064 - 46293577452674263141823442369649/664613997892457936451903530140172288))/9007199254740992 + sin(q3L)*((55491554575214198102159220722265*sin(q2L))/162259276829213363391578010288128 + cos(q2L)*((5557241208790345*cos(q1L))/9007199254740992 - (6384186990310915*sin(q1L))/9007199254740992) + (7514214926474921*sin(q2L)*((6384186990310915*cos(q1L))/9007199254740992 + (5557241208790345*sin(q1L))/9007199254740992))/36893488147419103232)))/36893488147419103232 + ((4503599440548691*cos(q4L))/4503599627370496 - (7514214926474921*sin(q4L))/36893488147419103232)*((7514214926474921*sin(q3L)*((55491554575214198102159220722265*cos(q2L))/162259276829213363391578010288128 + (7514214926474921*cos(q2L)*((6384186990310915*cos(q1L))/9007199254740992 + (5557241208790345*sin(q1L))/9007199254740992))/36893488147419103232 - sin(q2L)*((5557241208790345*cos(q1L))/9007199254740992 - (6384186990310915*sin(q1L))/9007199254740992)))/36893488147419103232 - cos(q3L)*((55491554575214198102159220722265*sin(q2L))/162259276829213363391578010288128 + cos(q2L)*((5557241208790345*cos(q1L))/9007199254740992 - (6384186990310915*sin(q1L))/9007199254740992) + (7514214926474921*sin(q2L)*((6384186990310915*cos(q1L))/9007199254740992 + (5557241208790345*sin(q1L))/9007199254740992))/36893488147419103232) + (9007199067919185*sin(q3L)*((57503643108550260546605243404275*cos(q1L))/81129638414606681695789005144064 + (50055177836018480443110068268825*sin(q1L))/81129638414606681695789005144064 - 46293577452674263141823442369649/664613997892457936451903530140172288))/9007199254740992) + ((234819211581865*cos(q4L))/1152921504606846976 + (9007199067919185*sin(q4L))/9007199254740992)*((432094733372955093709245836907320566011451687275*cos(q1L))/2993155353253689176481146537402947624255349848014848 - (499823478647255911063139966257565597426350154025*cos(q2L))/1461501637330902918203684832716283019655932542976 + (376125364442766701270516501597006072214248637825*sin(q1L))/2993155353253689176481146537402947624255349848014848 - (67682029681889335677290557259385*cos(q2L)*((6384186990310915*cos(q1L))/9007199254740992 + (5557241208790345*sin(q1L))/9007199254740992))/332306998946228968225951765070086144 + (9007199067919185*sin(q2L)*((5557241208790345*cos(q1L))/9007199254740992 - (6384186990310915*sin(q1L))/9007199254740992))/9007199254740992 - 347859890694807798813742879236295256254610072729/24519928653854221733733552434404946937899825954937634816)))/66461399789245793645190353014017228800 + (712008244765680093343103025701132101054572137019*cos(q5L)*((7514214926474921*sin(q4L)*((7514214926474921*cos(q3L)*((55491554575214198102159220722265*cos(q2L))/162259276829213363391578010288128 + (7514214926474921*cos(q2L)*((6384186990310915*cos(q1L))/9007199254740992 + (5557241208790345*sin(q1L))/9007199254740992))/36893488147419103232 - sin(q2L)*((5557241208790345*cos(q1L))/9007199254740992 - (6384186990310915*sin(q1L))/9007199254740992)))/36893488147419103232 + (9007199067919185*cos(q3L)*((57503643108550260546605243404275*cos(q1L))/81129638414606681695789005144064 + (50055177836018480443110068268825*sin(q1L))/81129638414606681695789005144064 - 46293577452674263141823442369649/664613997892457936451903530140172288))/9007199254740992 + sin(q3L)*((55491554575214198102159220722265*sin(q2L))/162259276829213363391578010288128 + cos(q2L)*((5557241208790345*cos(q1L))/9007199254740992 - (6384186990310915*sin(q1L))/9007199254740992) + (7514214926474921*sin(q2L)*((6384186990310915*cos(q1L))/9007199254740992 + (5557241208790345*sin(q1L))/9007199254740992))/36893488147419103232)))/36893488147419103232 + ((7514214926474921*cos(q4L))/36893488147419103232 + (4503599440548691*sin(q4L))/4503599627370496)*((7514214926474921*sin(q3L)*((55491554575214198102159220722265*cos(q2L))/162259276829213363391578010288128 + (7514214926474921*cos(q2L)*((6384186990310915*cos(q1L))/9007199254740992 + (5557241208790345*sin(q1L))/9007199254740992))/36893488147419103232 - sin(q2L)*((5557241208790345*cos(q1L))/9007199254740992 - (6384186990310915*sin(q1L))/9007199254740992)))/36893488147419103232 - cos(q3L)*((55491554575214198102159220722265*sin(q2L))/162259276829213363391578010288128 + cos(q2L)*((5557241208790345*cos(q1L))/9007199254740992 - (6384186990310915*sin(q1L))/9007199254740992) + (7514214926474921*sin(q2L)*((6384186990310915*cos(q1L))/9007199254740992 + (5557241208790345*sin(q1L))/9007199254740992))/36893488147419103232) + (9007199067919185*sin(q3L)*((57503643108550260546605243404275*cos(q1L))/81129638414606681695789005144064 + (50055177836018480443110068268825*sin(q1L))/81129638414606681695789005144064 - 46293577452674263141823442369649/664613997892457936451903530140172288))/9007199254740992) - ((9007199067919185*cos(q4L))/9007199254740992 - (234819211581865*sin(q4L))/1152921504606846976)*((432094733372955093709245836907320566011451687275*cos(q1L))/2993155353253689176481146537402947624255349848014848 - (499823478647255911063139966257565597426350154025*cos(q2L))/1461501637330902918203684832716283019655932542976 + (376125364442766701270516501597006072214248637825*sin(q1L))/2993155353253689176481146537402947624255349848014848 - (67682029681889335677290557259385*cos(q2L)*((6384186990310915*cos(q1L))/9007199254740992 + (5557241208790345*sin(q1L))/9007199254740992))/332306998946228968225951765070086144 + (9007199067919185*sin(q2L)*((5557241208790345*cos(q1L))/9007199254740992 - (6384186990310915*sin(q1L))/9007199254740992))/9007199254740992 - 347859890694807798813742879236295256254610072729/24519928653854221733733552434404946937899825954937634816)))/2451992865385422173373355243440494693789982595493763481600 + (81*((4503599440548691*cos(q4L))/4503599627370496 - (7514214926474921*sin(q4L))/36893488147419103232)*((7514214926474921*sin(q3L)*((55491554575214198102159220722265*cos(q2L))/162259276829213363391578010288128 + (7514214926474921*cos(q2L)*((6384186990310915*cos(q1L))/9007199254740992 + (5557241208790345*sin(q1L))/9007199254740992))/36893488147419103232 - sin(q2L)*((5557241208790345*cos(q1L))/9007199254740992 - (6384186990310915*sin(q1L))/9007199254740992)))/36893488147419103232 - cos(q3L)*((55491554575214198102159220722265*sin(q2L))/162259276829213363391578010288128 + cos(q2L)*((5557241208790345*cos(q1L))/9007199254740992 - (6384186990310915*sin(q1L))/9007199254740992) + (7514214926474921*sin(q2L)*((6384186990310915*cos(q1L))/9007199254740992 + (5557241208790345*sin(q1L))/9007199254740992))/36893488147419103232) + (9007199067919185*sin(q3L)*((57503643108550260546605243404275*cos(q1L))/81129638414606681695789005144064 + (50055177836018480443110068268825*sin(q1L))/81129638414606681695789005144064 - 46293577452674263141823442369649/664613997892457936451903530140172288))/9007199254740992))/2000 - (81222263116692158804177042061221826384594597321566869716687*((7514214926474921*cos(q4L))/36893488147419103232 + (4503599440548691*sin(q4L))/4503599627370496)*((7514214926474921*sin(q3L)*((55491554575214198102159220722265*cos(q2L))/162259276829213363391578010288128 + (7514214926474921*cos(q2L)*((6384186990310915*cos(q1L))/9007199254740992 + (5557241208790345*sin(q1L))/9007199254740992))/36893488147419103232 - sin(q2L)*((5557241208790345*cos(q1L))/9007199254740992 - (6384186990310915*sin(q1L))/9007199254740992)))/36893488147419103232 - cos(q3L)*((55491554575214198102159220722265*sin(q2L))/162259276829213363391578010288128 + cos(q2L)*((5557241208790345*cos(q1L))/9007199254740992 - (6384186990310915*sin(q1L))/9007199254740992) + (7514214926474921*sin(q2L)*((6384186990310915*cos(q1L))/9007199254740992 + (5557241208790345*sin(q1L))/9007199254740992))/36893488147419103232) + (9007199067919185*sin(q3L)*((57503643108550260546605243404275*cos(q1L))/81129638414606681695789005144064 + (50055177836018480443110068268825*sin(q1L))/81129638414606681695789005144064 - 46293577452674263141823442369649/664613997892457936451903530140172288))/9007199254740992))/306499108173177771671669405430061836723747824436720435200000 - (202883803014822867*sin(q5L)*((7514214926474921*sin(q4L)*((7514214926474921*cos(q3L)*((55491554575214198102159220722265*cos(q2L))/162259276829213363391578010288128 + (7514214926474921*cos(q2L)*((6384186990310915*cos(q1L))/9007199254740992 + (5557241208790345*sin(q1L))/9007199254740992))/36893488147419103232 - sin(q2L)*((5557241208790345*cos(q1L))/9007199254740992 - (6384186990310915*sin(q1L))/9007199254740992)))/36893488147419103232 + (9007199067919185*cos(q3L)*((57503643108550260546605243404275*cos(q1L))/81129638414606681695789005144064 + (50055177836018480443110068268825*sin(q1L))/81129638414606681695789005144064 - 46293577452674263141823442369649/664613997892457936451903530140172288))/9007199254740992 + sin(q3L)*((55491554575214198102159220722265*sin(q2L))/162259276829213363391578010288128 + cos(q2L)*((5557241208790345*cos(q1L))/9007199254740992 - (6384186990310915*sin(q1L))/9007199254740992) + (7514214926474921*sin(q2L)*((6384186990310915*cos(q1L))/9007199254740992 + (5557241208790345*sin(q1L))/9007199254740992))/36893488147419103232)))/36893488147419103232 + ((7514214926474921*cos(q4L))/36893488147419103232 + (4503599440548691*sin(q4L))/4503599627370496)*((7514214926474921*sin(q3L)*((55491554575214198102159220722265*cos(q2L))/162259276829213363391578010288128 + (7514214926474921*cos(q2L)*((6384186990310915*cos(q1L))/9007199254740992 + (5557241208790345*sin(q1L))/9007199254740992))/36893488147419103232 - sin(q2L)*((5557241208790345*cos(q1L))/9007199254740992 - (6384186990310915*sin(q1L))/9007199254740992)))/36893488147419103232 - cos(q3L)*((55491554575214198102159220722265*sin(q2L))/162259276829213363391578010288128 + cos(q2L)*((5557241208790345*cos(q1L))/9007199254740992 - (6384186990310915*sin(q1L))/9007199254740992) + (7514214926474921*sin(q2L)*((6384186990310915*cos(q1L))/9007199254740992 + (5557241208790345*sin(q1L))/9007199254740992))/36893488147419103232) + (9007199067919185*sin(q3L)*((57503643108550260546605243404275*cos(q1L))/81129638414606681695789005144064 + (50055177836018480443110068268825*sin(q1L))/81129638414606681695789005144064 - 46293577452674263141823442369649/664613997892457936451903530140172288))/9007199254740992) - ((9007199067919185*cos(q4L))/9007199254740992 - (234819211581865*sin(q4L))/1152921504606846976)*((432094733372955093709245836907320566011451687275*cos(q1L))/2993155353253689176481146537402947624255349848014848 - (499823478647255911063139966257565597426350154025*cos(q2L))/1461501637330902918203684832716283019655932542976 + (376125364442766701270516501597006072214248637825*sin(q1L))/2993155353253689176481146537402947624255349848014848 - (67682029681889335677290557259385*cos(q2L)*((6384186990310915*cos(q1L))/9007199254740992 + (5557241208790345*sin(q1L))/9007199254740992))/332306998946228968225951765070086144 + 